simulink library "outp"  (R2021b)
(part 7 of 10)

      link override Signal_Override/_ovrdflg: Value=KOUTP_RUNTM_s_ovrdflg
      link override Signal_Override/_ovrdval: Value=KOUTP_RUNTM_s_ovrdval
  VDID_ResetCDEODTR_km_Inproc : FVT_lib/outp/OverrideAndLimit  SystemSampleTime=-1  VariantActivationTime=update diagram  Latency=0  AutoFrameSizeCalculation=off
      link override Signal_Limit/_maxval: Value=KOUTP_ResetCDEODTR_km_maxval
      link override Signal_Limit/_minval: Value=KOUTP_ResetCDEODTR_km_minval
      link override Signal_Override/_ovrdflg: Value=KOUTP_ResetCDEODTR_km_ovrdflg
      link override Signal_Override/_ovrdval: Value=KOUTP_ResetCDEODTR_km_ovrdval
  VDID_STASUP_enum_Inproc : FVT_lib/outp/OverrideAndLimit  SystemSampleTime=-1  VariantActivationTime=update diagram  Latency=0  AutoFrameSizeCalculation=off
      link override Signal_Limit/_maxval: Value=KOUTP_STASUP_enum_maxval
      link override Signal_Limit/_minval: Value=KOUTP_STASUP_enum_minval
      link override Signal_Override/_ovrdflg: Value=KOUTP_STASUP_enum_ovrdflg
      link override Signal_Override/_ovrdval: Value=KOUTP_STASUP_enum_ovrdval
  VDID_TEBPSAL_kWh_Inproc : FVT_lib/outp/OverrideAndLimit  SystemSampleTime=-1  VariantActivationTime=update diagram  Latency=0  AutoFrameSizeCalculation=off
      link override Signal_Limit/_maxval: Value=KOUTP_TEBPSAL_kWh_maxval
      link override Signal_Limit/_minval: Value=KOUTP_TEBPSAL_kWh_minval
      link override Signal_Override/_ovrdflg: Value=KOUTP_TEBPSAL_kWh_ovrdflg
      link override Signal_Override/_ovrdval: Value=KOUTP_TEBPSAL_kWh_ovrdval
  VDID_TEBPSAR_kWh_Inproc : FVT_lib/outp/OverrideAndLimit  SystemSampleTime=-1  VariantActivationTime=update diagram  Latency=0  AutoFrameSizeCalculation=off
      link override Signal_Limit/_maxval: Value=KOUTP_TEBPSAR_kWh_maxval
      link override Signal_Limit/_minval: Value=KOUTP_TEBPSAR_kWh_minval
      link override Signal_Override/_ovrdflg: Value=KOUTP_TEBPSAR_kWh_ovrdflg
      link override Signal_Override/_ovrdval: Value=KOUTP_TEBPSAR_kWh_ovrdval
  VDID_TGEOVCL_kWh_Inproc : FVT_lib/outp/OverrideAndLimit  SystemSampleTime=-1  VariantActivationTime=update diagram  Latency=0  AutoFrameSizeCalculation=off
      link override Signal_Limit/_maxval: Value=KOUTP_TGEOVCL_kWh_maxval
      link override Signal_Limit/_minval: Value=KOUTP_TGEOVCL_kWh_minval
      link override Signal_Override/_ovrdflg: Value=KOUTP_TGEOVCL_kWh_ovrdflg
      link override Signal_Override/_ovrdval: Value=KOUTP_TGEOVCL_kWh_ovrdval
  VDID_TGEOVCR_kWh_Inproc : FVT_lib/outp/OverrideAndLimit  SystemSampleTime=-1  VariantActivationTime=update diagram  Latency=0  AutoFrameSizeCalculation=off
      link override Signal_Limit/_maxval: Value=KOUTP_TGEOVCR_kWh_maxval
      link override Signal_Limit/_minval: Value=KOUTP_TGEOVCR_kWh_minval
      link override Signal_Override/_ovrdflg: Value=KOUTP_TGEOVCR_kWh_ovrdflg
      link override Signal_Override/_ovrdval: Value=KOUTP_TGEOVCR_kWh_ovrdval
  VDID_TNBCPSAL_Ahr_Inproc : FVT_lib/outp/OverrideAndLimit  SystemSampleTime=-1  VariantActivationTime=update diagram  Latency=0  AutoFrameSizeCalculation=off
      link override Signal_Limit/_maxval: Value=KOUTP_TNBCPSAL_Ahr_maxval
      link override Signal_Limit/_minval: Value=KOUTP_TNBCPSAL_Ahr_minval
      link override Signal_Override/_ovrdflg: Value=KOUTP_TNBCPSAL_Ahr_ovrdflg
      link override Signal_Override/_ovrdval: Value=KOUTP_TNBCPSAL_Ahr_ovrdval
  VDID_TNBCPSAR_Ahr_Inproc : FVT_lib/outp/OverrideAndLimit  SystemSampleTime=-1  VariantActivationTime=update diagram  Latency=0  AutoFrameSizeCalculation=off
      link override Signal_Limit/_maxval: Value=KOUTP_TNBCPSAR_Ahr_maxval
      link override Signal_Limit/_minval: Value=KOUTP_TNBCPSAR_Ahr_minval
      link override Signal_Override/_ovrdflg: Value=KOUTP_TNBCPSAR_Ahr_ovrdflg
      link override Signal_Override/_ovrdval: Value=KOUTP_TNBCPSAR_Ahr_ovrdval
  VDID_TNECPSAL_kWh_Inproc : FVT_lib/outp/OverrideAndLimit  SystemSampleTime=-1  VariantActivationTime=update diagram  Latency=0  AutoFrameSizeCalculation=off
      link override Signal_Limit/_maxval: Value=KOUTP_TNECPSAL_kWh_maxval
      link override Signal_Limit/_minval: Value=KOUTP_TNECPSAL_kWh_minval
      link override Signal_Override/_ovrdflg: Value=KOUTP_TNECPSAL_kWh_ovrdflg
      link override Signal_Override/_ovrdval: Value=KOUTP_TNECPSAL_kWh_ovrdval
  VDID_TNECPSAR_kWh_Inproc : FVT_lib/outp/OverrideAndLimit  SystemSampleTime=-1  VariantActivationTime=update diagram  Latency=0  AutoFrameSizeCalculation=off
      link override Signal_Limit/_maxval: Value=KOUTP_TNECPSAR_kWh_maxval
      link override Signal_Limit/_minval: Value=KOUTP_TNECPSAR_kWh_minval
      link override Signal_Override/_ovrdflg: Value=KOUTP_TNECPSAR_kWh_ovrdflg
      link override Signal_Override/_ovrdval: Value=KOUTP_TNECPSAR_kWh_ovrdval
  VDID_VSS_kph_Inproc : FVT_lib/outp/OverrideAndLimit  SystemSampleTime=-1  VariantActivationTime=update diagram  Latency=0  AutoFrameSizeCalculation=off
      link override Signal_Limit/_maxval: Value=KOUTP_VSS_kph_maxval
      link override Signal_Limit/_minval: Value=KOUTP_VSS_kph_minval
      link override Signal_Override/_ovrdflg: Value=KOUTP_VSS_kph_ovrdflg
      link override Signal_Override/_ovrdval: Value=KOUTP_VSS_kph_ovrdval
  VDID_VinCode_cnt_Inproc : FVT_lib/outp/OverrideAndLimit  SystemSampleTime=-1  VariantActivationTime=update diagram  Latency=0  AutoFrameSizeCalculation=off
      link override Signal_Limit/_maxval: Value=KOUTP_VinCode_cnt_maxval
      link override Signal_Limit/_minval: Value=KOUTP_VinCode_cnt_minval
      link override Signal_Override/_ovrdflg: Value=KOUTP_VinCode_cnt_ovrdflg
      link override Signal_Override/_ovrdval: Value=KOUTP_VinCode_cnt_ovrdval
  VDID_WARMUPS_cnt_Inproc : FVT_lib/outp/OverrideAndLimit  SystemSampleTime=-1  VariantActivationTime=update diagram  Latency=0  AutoFrameSizeCalculation=off
      link override Signal_Limit/_maxval: Value=KOUTP_WARMUPS_cnt_maxval
      link override Signal_Limit/_minval: Value=KOUTP_WARMUPS_cnt_minval
      link override Signal_Override/_ovrdflg: Value=KOUTP_WARMUPS_cnt_ovrdflg
      link override Signal_Override/_ovrdval: Value=KOUTP_WARMUPS_cnt_ovrdval
  VDKC_DKCAuthSta_enum_Inproc : FVT_lib/outp/OverrideAndLimit  SystemSampleTime=-1  VariantActivationTime=update diagram  Latency=0  AutoFrameSizeCalculation=off
      link override Signal_Limit/_maxval: Value=KOUTP_DKCAuthSta_enum_maxval
      link override Signal_Limit/_minval: Value=KOUTP_DKCAuthSta_enum_minval
      link override Signal_Override/_ovrdflg: Value=KOUTP_DKCAuthSta_enum_ovrdflg
      link override Signal_Override/_ovrdval: Value=KOUTP_DKCAuthSta_enum_ovrdval
  VDKC_DKCTimeSN_cnt_Inproc : FVT_lib/outp/OverrideAndLimit  SystemSampleTime=-1  VariantActivationTime=update diagram  Latency=0  AutoFrameSizeCalculation=off
      link override Signal_Limit/_maxval: Value=KOUTP_DKCTimeSN_cnt_maxval
      link override Signal_Limit/_minval: Value=KOUTP_DKCTimeSN_cnt_minval
      link override Signal_Override/_ovrdflg: Value=KOUTP_DKCTimeSN_cnt_ovrdflg
      link override Signal_Override/_ovrdval: Value=KOUTP_DKCTimeSN_cnt_ovrdval
  VDKC_DKeyWelcomeSta_enum_Inproc : FVT_lib/outp/OverrideAndLimit  SystemSampleTime=-1  VariantActivationTime=update diagram  Latency=0  AutoFrameSizeCalculation=off
      link override Signal_Limit/_maxval: Value=KOUTP_DKeyWelcomeSta_enum_maxval
      link override Signal_Limit/_minval: Value=KOUTP_DKeyWelcomeSta_enum_minval
      link override Signal_Override/_ovrdflg: Value=KOUTP_DKeyWelcomeSta_enum_ovrdflg
      link override Signal_Override/_ovrdval: Value=KOUTP_DKeyWelcomeSta_enum_ovrdval
  VDKC_DkeyAreaRAPSSta_enum_Inproc : FVT_lib/outp/OverrideAndLimit  SystemSampleTime=-1  VariantActivationTime=update diagram  Latency=0  AutoFrameSizeCalculation=off
      link override Signal_Limit/_maxval: Value=KOUTP_DkeyAreaRAPSSta_enum_maxval
      link override Signal_Limit/_minval: Value=KOUTP_DkeyAreaRAPSSta_enum_minval
      link override Signal_Override/_ovrdflg: Value=KOUTP_DkeyAreaRAPSSta_enum_ovrdflg
      link override Signal_Override/_ovrdval: Value=KOUTP_DkeyAreaRAPSSta_enum_ovrdval
  VDKC_DkeyShowIVISta_enum_Inproc : FVT_lib/outp/OverrideAndLimit  SystemSampleTime=-1  VariantActivationTime=update diagram  Latency=0  AutoFrameSizeCalculation=off
      link override Signal_Limit/_maxval: Value=KOUTP_DkeyShowIVISta_enum_maxval
      link override Signal_Limit/_minval: Value=KOUTP_DkeyShowIVISta_enum_minval
      link override Signal_Override/_ovrdflg: Value=KOUTP_DkeyShowIVISta_enum_ovrdflg
      link override Signal_Override/_ovrdval: Value=KOUTP_DkeyShowIVISta_enum_ovrdval
  VDKC_FDCDKCAllowSleep_flg_Inproc : FVT_lib/outp/OverrideAndLimit  SystemSampleTime=-1  VariantActivationTime=update diagram  Latency=0  AutoFrameSizeCalculation=off
      link override Signal_Limit/_maxval: Value=KOUTP_FDCDKCAllowSleep_flg_maxval
      link override Signal_Limit/_minval: Value=KOUTP_FDCDKCAllowSleep_flg_minval
      link override Signal_Override/_ovrdflg: Value=KOUTP_FDCDKCAllowSleep_flg_ovrdflg
      link override Signal_Override/_ovrdval: Value=KOUTP_FDCDKCAllowSleep_flg_ovrdval
  VDKC_JudgeKeepUnlockZone_flg_Inproc : FVT_lib/outp/OverrideAndLimit  SystemSampleTime=-1  VariantActivationTime=update diagram  Latency=0  AutoFrameSizeCalculation=off
      link override Signal_Limit/_maxval: Value=KOUTP_JudgeKeepUnlockZone_flg_maxval
      link override Signal_Limit/_minval: Value=KOUTP_JudgeKeepUnlockZone_flg_minval
      link override Signal_Override/_ovrdflg: Value=KOUTP_JudgeKeepUnlockZone_flg_ovrdflg
      link override Signal_Override/_ovrdval: Value=KOUTP_JudgeKeepUnlockZone_flg_ovrdval
  VDKC_KeyAreaLockUnlock_enum_Inproc : FVT_lib/outp/OverrideAndLimit  SystemSampleTime=-1  VariantActivationTime=update diagram  Latency=0  AutoFrameSizeCalculation=off
      link override Signal_Limit/_maxval: Value=KOUTP_KeyAreaLockUnlock_enum_maxval
      link override Signal_Limit/_minval: Value=KOUTP_KeyAreaLockUnlock_enum_minval
      link override Signal_Override/_ovrdflg: Value=KOUTP_KeyAreaLockUnlock_enum_ovrdflg
      link override Signal_Override/_ovrdval: Value=KOUTP_KeyAreaLockUnlock_enum_ovrdval
  VDKC_KeyAreaPS_enum_Inproc : FVT_lib/outp/OverrideAndLimit  SystemSampleTime=-1  VariantActivationTime=update diagram  Latency=0  AutoFrameSizeCalculation=off
      link override Signal_Limit/_maxval: Value=KOUTP_KeyAreaPS_enum_maxval
      link override Signal_Limit/_minval: Value=KOUTP_KeyAreaPS_enum_minval
      link override Signal_Override/_ovrdflg: Value=KOUTP_KeyAreaPS_enum_ovrdflg
      link override Signal_Override/_ovrdval: Value=KOUTP_KeyAreaPS_enum_ovrdval
  VDKC_KeyAreaPTG_enum_Inproc : FVT_lib/outp/OverrideAndLimit  SystemSampleTime=-1  VariantActivationTime=update diagram  Latency=0  AutoFrameSizeCalculation=off
      link override Signal_Limit/_maxval: Value=KOUTP_KeyAreaPTG_enum_maxval
      link override Signal_Limit/_minval: Value=KOUTP_KeyAreaPTG_enum_minval
      link override Signal_Override/_ovrdflg: Value=KOUTP_KeyAreaPTG_enum_ovrdflg
      link override Signal_Override/_ovrdval: Value=KOUTP_KeyAreaPTG_enum_ovrdval
  VDKC_KeyAreaSPTGSta_enum_Inproc : FVT_lib/outp/OverrideAndLimit  SystemSampleTime=-1  VariantActivationTime=update diagram  Latency=0  AutoFrameSizeCalculation=off
      link override Signal_Limit/_maxval: Value=KOUTP_KeyAreaSPTGSta_enum_maxval
      link override Signal_Limit/_minval: Value=KOUTP_KeyAreaSPTGSta_enum_minval
      link override Signal_Override/_ovrdflg: Value=KOUTP_KeyAreaSPTGSta_enum_ovrdflg
      link override Signal_Override/_ovrdval: Value=KOUTP_KeyAreaSPTGSta_enum_ovrdval
  VDKC_KeyMissSta_flg_Inproc : FVT_lib/outp/OverrideAndLimit  SystemSampleTime=-1  VariantActivationTime=update diagram  Latency=0  AutoFrameSizeCalculation=off
      link override Signal_Limit/_maxval: Value=KOUTP_KeyMissSta_flg_maxval
      link override Signal_Limit/_minval: Value=KOUTP_KeyMissSta_flg_minval
      link override Signal_Override/_ovrdflg: Value=KOUTP_KeyMissSta_flg_ovrdflg
      link override Signal_Override/_ovrdval: Value=KOUTP_KeyMissSta_flg_ovrdval
  VDKC_KeyModeSta_enum_Inproc : FVT_lib/outp/OverrideAndLimit  SystemSampleTime=-1  VariantActivationTime=update diagram  Latency=0  AutoFrameSizeCalculation=off
      link override Signal_Limit/_maxval: Value=KOUTP_KeyModeSta_enum_maxval
      link override Signal_Limit/_minval: Value=KOUTP_KeyModeSta_enum_minval
      link override Signal_Override/_ovrdflg: Value=KOUTP_KeyModeSta_enum_ovrdflg
      link override Signal_Override/_ovrdval: Value=KOUTP_KeyModeSta_enum_ovrdval
  VDKC_KeyNumSta_enum_Inproc : FVT_lib/outp/OverrideAndLimit  SystemSampleTime=-1  VariantActivationTime=update diagram  Latency=0  AutoFrameSizeCalculation=off
      link override Signal_Limit/_maxval: Value=KOUTP_KeyNumSta_enum_maxval
      link override Signal_Limit/_minval: Value=KOUTP_KeyNumSta_enum_minval
      link override Signal_Override/_ovrdflg: Value=KOUTP_KeyNumSta_enum_ovrdflg
      link override Signal_Override/_ovrdval: Value=KOUTP_KeyNumSta_enum_ovrdval
  VDKC_KeyTypeSta_enum_Inproc : FVT_lib/outp/OverrideAndLimit  SystemSampleTime=-1  VariantActivationTime=update diagram  Latency=0  AutoFrameSizeCalculation=off
      link override Signal_Limit/_maxval: Value=KOUTP_KeyTypeSta_enum_maxval
      link override Signal_Limit/_minval: Value=KOUTP_KeyTypeSta_enum_minval
      link override Signal_Override/_ovrdflg: Value=KOUTP_KeyTypeSta_enum_ovrdflg
      link override Signal_Override/_ovrdval: Value=KOUTP_KeyTypeSta_enum_ovrdval
  VDKC_PCommandToBCM_enum_Inproc : FVT_lib/outp/OverrideAndLimit  SystemSampleTime=-1  VariantActivationTime=update diagram  Latency=0  AutoFrameSizeCalculation=off
      link override Signal_Limit/_maxval: Value=KOUTP_PCommandToBCM_enum_maxval
      link override Signal_Limit/_minval: Value=KOUTP_PCommandToBCM_enum_minval
      link override Signal_Override/_ovrdflg: Value=KOUTP_PCommandToBCM_enum_ovrdflg
      link override Signal_Override/_ovrdval: Value=KOUTP_PCommandToBCM_enum_ovrdval
  VDKC_ParkingModeCmd_enum_Inproc : FVT_lib/outp/OverrideAndLimit  SystemSampleTime=-1  VariantActivationTime=update diagram  Latency=0  AutoFrameSizeCalculation=off
      link override Signal_Limit/_maxval: Value=KOUTP_ParkingModeCmd_enum_maxval
      link override Signal_Limit/_minval: Value=KOUTP_ParkingModeCmd_enum_minval
      link override Signal_Override/_ovrdflg: Value=KOUTP_ParkingModeCmd_enum_ovrdflg
      link override Signal_Override/_ovrdval: Value=KOUTP_ParkingModeCmd_enum_ovrdval
  VDKC_TimeSNDKCFbk_cnt_Inproc : FVT_lib/outp/OverrideAndLimit  SystemSampleTime=-1  VariantActivationTime=update diagram  Latency=0  AutoFrameSizeCalculation=off
      link override Signal_Limit/_maxval: Value=KOUTP_TimeSNDKCFbk_cnt_maxval
      link override Signal_Limit/_minval: Value=KOUTP_TimeSNDKCFbk_cnt_minval
      link override Signal_Override/_ovrdflg: Value=KOUTP_TimeSNDKCFbk_cnt_ovrdflg
      link override Signal_Override/_ovrdval: Value=KOUTP_TimeSNDKCFbk_cnt_ovrdval
  VDKC_UIDLowPowerSta_enum_Inproc : FVT_lib/outp/OverrideAndLimit  SystemSampleTime=-1  VariantActivationTime=update diagram  Latency=0  AutoFrameSizeCalculation=off
      link override Signal_Limit/_maxval: Value=KOUTP_UIDLowPowerSta_enum_maxval
      link override Signal_Limit/_minval: Value=KOUTP_UIDLowPowerSta_enum_minval
      link override Signal_Override/_ovrdflg: Value=KOUTP_UIDLowPowerSta_enum_ovrdflg
      link override Signal_Override/_ovrdval: Value=KOUTP_UIDLowPowerSta_enum_ovrdval
  VDSC_DISCButtSta_flg_Inproc : FVT_lib/outp/OverrideAndLimit  SystemSampleTime=-1  VariantActivationTime=update diagram  Latency=0  AutoFrameSizeCalculation=off
      link override Signal_Limit/_maxval: Value=KOUTP_DISCButtSta_flg_maxval
      link override Signal_Limit/_minval: Value=KOUTP_DISCButtSta_flg_minval
      link override Signal_Override/_ovrdflg: Value=KOUTP_DISCButtSta_flg_ovrdflg
      link override Signal_Override/_ovrdval: Value=KOUTP_DISCButtSta_flg_ovrdval
  VDSC_DISCSta_enum_Inproc : FVT_lib/outp/OverrideAndLimit  SystemSampleTime=-1  VariantActivationTime=update diagram  Latency=0  AutoFrameSizeCalculation=off
      link override Signal_Limit/_maxval: Value=KOUTP_DISCSta_enum_maxval
      link override Signal_Limit/_minval: Value=KOUTP_DISCSta_enum_minval
      link override Signal_Override/_ovrdflg: Value=KOUTP_DISCSta_enum_ovrdflg
      link override Signal_Override/_ovrdval: Value=KOUTP_DISCSta_enum_ovrdval
  VDSC_DISCTargetSpd_kph_Inproc : FVT_lib/outp/OverrideAndLimit  SystemSampleTime=-1  VariantActivationTime=update diagram  Latency=0  AutoFrameSizeCalculation=off
      link override Signal_Limit/_maxval: Value=KOUTP_DISCTargetSpd_kph_maxval
      link override Signal_Limit/_minval: Value=KOUTP_DISCTargetSpd_kph_minval
      link override Signal_Override/_ovrdflg: Value=KOUTP_DISCTargetSpd_kph_ovrdflg
      link override Signal_Override/_ovrdval: Value=KOUTP_DISCTargetSpd_kph_ovrdval
  VDSC_DISCTurn_flg_Inproc : FVT_lib/outp/OverrideAndLimit  SystemSampleTime=-1  VariantActivationTime=update diagram  Latency=0  AutoFrameSizeCalculation=off
      link override Signal_Limit/_maxval: Value=KOUTP_DISCTurn_flg_maxval
      link override Signal_Limit/_minval: Value=KOUTP_DISCTurn_flg_minval
      link override Signal_Override/_ovrdflg: Value=KOUTP_DISCTurn_flg_ovrdflg
      link override Signal_Override/_ovrdval: Value=KOUTP_DISCTurn_flg_ovrdval
  VNMM_ActiveWU_flg_Inproc : FVT_lib/outp/OverrideAndLimit  SystemSampleTime=-1  VariantActivationTime=update diagram  Latency=0  AutoFrameSizeCalculation=off
      link override Signal_Limit/_maxval: Value=KOUTP_ActiveWU_flg_maxval
      link override Signal_Limit/_minval: Value=KOUTP_ActiveWU_flg_minval
      link override Signal_Override/_ovrdflg: Value=KOUTP_ActiveWU_flg_ovrdflg
      link override Signal_Override/_ovrdval: Value=KOUTP_ActiveWU_flg_ovrdval
  VNMM_AllCANTxReq_flg_Inproc : FVT_lib/outp/OverrideAndLimit  SystemSampleTime=-1  VariantActivationTime=update diagram  Latency=0  AutoFrameSizeCalculation=off
      link override Signal_Limit/_maxval: Value=KOUTP_AllCANTxReq_flg_maxval
      link override Signal_Limit/_minval: Value=KOUTP_AllCANTxReq_flg_minval
      link override Signal_Override/_ovrdflg: Value=KOUTP_AllCANTxReq_flg_ovrdflg
      link override Signal_Override/_ovrdval: Value=KOUTP_AllCANTxReq_flg_ovrdval
  VNMM_Awake_enum_Inproc : FVT_lib/outp/OverrideAndLimit  SystemSampleTime=-1  VariantActivationTime=update diagram  Latency=0  AutoFrameSizeCalculation=off
      link override Signal_Limit/_maxval: Value=KOUTP_Awake_enum_maxval
      link override Signal_Limit/_minval: Value=KOUTP_Awake_enum_minval
      link override Signal_Override/_ovrdflg: Value=KOUTP_Awake_enum_ovrdflg
      link override Signal_Override/_ovrdval: Value=KOUTP_Awake_enum_ovrdval
  VNMM_CSB_flg_Inproc : FVT_lib/outp/OverrideAndLimit  SystemSampleTime=-1  VariantActivationTime=update diagram  Latency=0  AutoFrameSizeCalculation=off
      link override Signal_Limit/_maxval: Value=KOUTP_CSB_flg_maxval
      link override Signal_Limit/_minval: Value=KOUTP_CSB_flg_minval
      link override Signal_Override/_ovrdflg: Value=KOUTP_CSB_flg_ovrdflg
      link override Signal_Override/_ovrdval: Value=KOUTP_CSB_flg_ovrdval
  VNMM_ErrorState_enum_Inproc : FVT_lib/outp/OverrideAndLimit  SystemSampleTime=-1  VariantActivationTime=update diagram  Latency=0  AutoFrameSizeCalculation=off
      link override Signal_Limit/_maxval: Value=KOUTP_ErrorState_enum_maxval
      link override Signal_Limit/_minval: Value=KOUTP_ErrorState_enum_minval
      link override Signal_Override/_ovrdflg: Value=KOUTP_ErrorState_enum_ovrdflg
      link override Signal_Override/_ovrdval: Value=KOUTP_ErrorState_enum_ovrdval
  VNMM_NMmTxReq_flg_Inproc : FVT_lib/outp/OverrideAndLimit  SystemSampleTime=-1  VariantActivationTime=update diagram  Latency=0  AutoFrameSizeCalculation=off
      link override Signal_Limit/_maxval: Value=KOUTP_NMmTxReq_flg_maxval
      link override Signal_Limit/_minval: Value=KOUTP_NMmTxReq_flg_minval
      link override Signal_Override/_ovrdflg: Value=KOUTP_NMmTxReq_flg_ovrdflg
      link override Signal_Override/_ovrdval: Value=KOUTP_NMmTxReq_flg_ovrdval
  VNMM_NetworkReq_flg_Inproc : FVT_lib/outp/OverrideAndLimit  SystemSampleTime=-1  VariantActivationTime=update diagram  Latency=0  AutoFrameSizeCalculation=off
      link override Signal_Limit/_maxval: Value=KOUTP_NetworkReq_flg_maxval
      link override Signal_Limit/_minval: Value=KOUTP_NetworkReq_flg_minval
      link override Signal_Override/_ovrdflg: Value=KOUTP_NetworkReq_flg_ovrdflg
      link override Signal_Override/_ovrdval: Value=KOUTP_NetworkReq_flg_ovrdval
  VNMM_NodeID_enum_Inproc : FVT_lib/outp/OverrideAndLimit  SystemSampleTime=-1  VariantActivationTime=update diagram  Latency=0  AutoFrameSizeCalculation=off
      link override Signal_Limit/_maxval: Value=KOUTP_NodeID_enum_maxval
      link override Signal_Limit/_minval: Value=KOUTP_NodeID_enum_minval
      link override Signal_Override/_ovrdflg: Value=KOUTP_NodeID_enum_ovrdflg
      link override Signal_Override/_ovrdval: Value=KOUTP_NodeID_enum_ovrdval
  VNMM_PNI_flg_Inproc : FVT_lib/outp/OverrideAndLimit  SystemSampleTime=-1  VariantActivationTime=update diagram  Latency=0  AutoFrameSizeCalculation=off
      link override Signal_Limit/_maxval: Value=KOUTP_PNI_flg_maxval
      link override Signal_Limit/_minval: Value=KOUTP_PNI_flg_minval
      link override Signal_Override/_ovrdflg: Value=KOUTP_PNI_flg_ovrdflg
      link override Signal_Override/_ovrdval: Value=KOUTP_PNI_flg_ovrdval
  VNMM_RptMsgReq_flg_Inproc : FVT_lib/outp/OverrideAndLimit  SystemSampleTime=-1  VariantActivationTime=update diagram  Latency=0  AutoFrameSizeCalculation=off
      link override Signal_Limit/_maxval: Value=KOUTP_RptMsgReq_flg_maxval
      link override Signal_Limit/_minval: Value=KOUTP_RptMsgReq_flg_minval
      link override Signal_Override/_ovrdflg: Value=KOUTP_RptMsgReq_flg_ovrdflg
      link override Signal_Override/_ovrdval: Value=KOUTP_RptMsgReq_flg_ovrdval
  VNMM_SysNMmSta_enum_Inproc : FVT_lib/outp/OverrideAndLimit  SystemSampleTime=-1  VariantActivationTime=update diagram  Latency=0  AutoFrameSizeCalculation=off
      link override Signal_Limit/_maxval: Value=KOUTP_SysNMmSta_enum_maxval
      link override Signal_Limit/_minval: Value=KOUTP_SysNMmSta_enum_minval
      link override Signal_Override/_ovrdflg: Value=KOUTP_SysNMmSta_enum_ovrdflg
      link override Signal_Override/_ovrdval: Value=KOUTP_SysNMmSta_enum_ovrdval
  VNMM_WakeUp_enum_Inproc : FVT_lib/outp/OverrideAndLimit  SystemSampleTime=-1  VariantActivationTime=update diagram  Latency=0  AutoFrameSizeCalculation=off
      link override Signal_Limit/_maxval: Value=KOUTP_WakeUp_enum_maxval
      link override Signal_Limit/_minval: Value=KOUTP_WakeUp_enum_minval
      link override Signal_Override/_ovrdflg: Value=KOUTP_WakeUp_enum_ovrdflg
      link override Signal_Override/_ovrdval: Value=KOUTP_WakeUp_enum_ovrdval
  VPMM_ACHVLoopDem_enum_Inproc : FVT_lib/outp/OverrideAndLimit  SystemSampleTime=-1  VariantActivationTime=update diagram  Latency=0  AutoFrameSizeCalculation=off
      link override Signal_Limit/_maxval: Value=KOUTP_ACHVLoopDem_enum_maxval
      link override Signal_Limit/_minval: Value=KOUTP_ACHVLoopDem_enum_minval
      link override Signal_Override/_ovrdflg: Value=KOUTP_ACHVLoopDem_enum_ovrdflg
      link override Signal_Override/_ovrdval: Value=KOUTP_ACHVLoopDem_enum_ovrdval
  VPMM_ActiveDischargeReq_enum_Inproc : FVT_lib/outp/OverrideAndLimit  SystemSampleTime=-1  VariantActivationTime=update diagram  Latency=0  AutoFrameSizeCalculation=off
      link override Signal_Limit/_maxval: Value=KOUTP_ActiveDischargeReq_enum_maxval
      link override Signal_Limit/_minval: Value=KOUTP_ActiveDischargeReq_enum_minval
      link override Signal_Override/_ovrdflg: Value=KOUTP_ActiveDischargeReq_enum_ovrdflg
      link override Signal_Override/_ovrdval: Value=KOUTP_ActiveDischargeReq_enum_ovrdval
  VPMM_BattHVDem_enum_Inproc : FVT_lib/outp/OverrideAndLimit  SystemSampleTime=-1  VariantActivationTime=update diagram  Latency=0  AutoFrameSizeCalculation=off
      link override Signal_Limit/_maxval: Value=KOUTP_BattHVDem_enum_maxval
      link override Signal_Limit/_minval: Value=KOUTP_BattHVDem_enum_minval
      link override Signal_Override/_ovrdflg: Value=KOUTP_BattHVDem_enum_ovrdflg
      link override Signal_Override/_ovrdval: Value=KOUTP_BattHVDem_enum_ovrdval
  VPMM_CACRlyDem_enum_Inproc : FVT_lib/outp/OverrideAndLimit  SystemSampleTime=-1  VariantActivationTime=update diagram  Latency=0  AutoFrameSizeCalculation=off
      link override Signal_Limit/_maxval: Value=KOUTP_CACRlyDem_enum_maxval
      link override Signal_Limit/_minval: Value=KOUTP_CACRlyDem_enum_minval
      link override Signal_Override/_ovrdflg: Value=KOUTP_CACRlyDem_enum_ovrdflg
      link override Signal_Override/_ovrdval: Value=KOUTP_CACRlyDem_enum_ovrdval
  VPMM_ChrgBCUHVFail_flg_Inproc : FVT_lib/outp/OverrideAndLimit  SystemSampleTime=-1  VariantActivationTime=update diagram  Latency=0  AutoFrameSizeCalculation=off
      link override Signal_Limit/_maxval: Value=KOUTP_ChrgBCUHVFail_flg_maxval
      link override Signal_Limit/_minval: Value=KOUTP_ChrgBCUHVFail_flg_minval
      link override Signal_Override/_ovrdflg: Value=KOUTP_ChrgBCUHVFail_flg_ovrdflg
      link override Signal_Override/_ovrdval: Value=KOUTP_ChrgBCUHVFail_flg_ovrdval
  VPMM_ChrgFault_enum_Inproc : FVT_lib/outp/OverrideAndLimit  SystemSampleTime=-1  VariantActivationTime=update diagram  Latency=0  AutoFrameSizeCalculation=off
      link override Signal_Limit/_maxval: Value=KOUTP_ChrgFault_enum_maxval
      link override Signal_Limit/_minval: Value=KOUTP_ChrgFault_enum_minval
      link override Signal_Override/_ovrdflg: Value=KOUTP_ChrgFault_enum_ovrdflg
      link override Signal_Override/_ovrdval: Value=KOUTP_ChrgFault_enum_ovrdval
  VPMM_ChrgPowerUpFail_flg_Inproc : FVT_lib/outp/OverrideAndLimit  SystemSampleTime=-1  VariantActivationTime=update diagram  Latency=0  AutoFrameSizeCalculation=off
      link override Signal_Limit/_maxval: Value=KOUTP_ChrgPowerUpFail_flg_maxval
      link override Signal_Limit/_minval: Value=KOUTP_ChrgPowerUpFail_flg_minval
      link override Signal_Override/_ovrdflg: Value=KOUTP_ChrgPowerUpFail_flg_ovrdflg
      link override Signal_Override/_ovrdval: Value=KOUTP_ChrgPowerUpFail_flg_ovrdval
  VPMM_ChrgState_enum_Inproc : FVT_lib/outp/OverrideAndLimit  SystemSampleTime=-1  VariantActivationTime=update diagram  Latency=0  AutoFrameSizeCalculation=off
      link override Signal_Limit/_maxval: Value=KOUTP_ChrgState_enum_maxval
      link override Signal_Limit/_minval: Value=KOUTP_ChrgState_enum_minval
      link override Signal_Override/_ovrdflg: Value=KOUTP_ChrgState_enum_ovrdflg
      link override Signal_Override/_ovrdval: Value=KOUTP_ChrgState_enum_ovrdval
  VPMM_DCCurr_A_Inproc : FVT_lib/outp/OverrideAndLimit  SystemSampleTime=-1  VariantActivationTime=update diagram  Latency=0  AutoFrameSizeCalculation=off
      link override Signal_Limit/_maxval: Value=KOUTP_DCCurr_A_maxval
      link override Signal_Limit/_minval: Value=KOUTP_DCCurr_A_minval
      link override Signal_Override/_ovrdflg: Value=KOUTP_DCCurr_A_ovrdflg
      link override Signal_Override/_ovrdval: Value=KOUTP_DCCurr_A_ovrdval
  VPMM_DCDCRlyDem_enum_Inproc : FVT_lib/outp/OverrideAndLimit  SystemSampleTime=-1  VariantActivationTime=update diagram  Latency=0  AutoFrameSizeCalculation=off
      link override Signal_Limit/_maxval: Value=KOUTP_DCDCRlyDem_enum_maxval
      link override Signal_Limit/_minval: Value=KOUTP_DCDCRlyDem_enum_minval
      link override Signal_Override/_ovrdflg: Value=KOUTP_DCDCRlyDem_enum_ovrdflg
      link override Signal_Override/_ovrdval: Value=KOUTP_DCDCRlyDem_enum_ovrdval
  VPMM_DCVol_V_Inproc : FVT_lib/outp/OverrideAndLimit  SystemSampleTime=-1  VariantActivationTime=update diagram  Latency=0  AutoFrameSizeCalculation=off
      link override Signal_Limit/_maxval: Value=KOUTP_DCVol_V_maxval
      link override Signal_Limit/_minval: Value=KOUTP_DCVol_V_minval
      link override Signal_Override/_ovrdflg: Value=KOUTP_DCVol_V_ovrdflg
      link override Signal_Override/_ovrdval: Value=KOUTP_DCVol_V_ovrdval
  VPMM_DrivelineRelease_enum_Inproc : FVT_lib/outp/OverrideAndLimit  SystemSampleTime=-1  VariantActivationTime=update diagram  Latency=0  AutoFrameSizeCalculation=off
      link override Signal_Limit/_maxval: Value=KOUTP_DrivelineRelease_enum_maxval
      link override Signal_Limit/_minval: Value=KOUTP_DrivelineRelease_enum_minval
      link override Signal_Override/_ovrdflg: Value=KOUTP_DrivelineRelease_enum_ovrdflg
      link override Signal_Override/_ovrdval: Value=KOUTP_DrivelineRelease_enum_ovrdval
  VPMM_EHPSRlyDem_enum_Inproc : FVT_lib/outp/OverrideAndLimit  SystemSampleTime=-1  VariantActivationTime=update diagram  Latency=0  AutoFrameSizeCalculation=off
      link override Signal_Limit/_maxval: Value=KOUTP_EHPSRlyDem_enum_maxval
      link override Signal_Limit/_minval: Value=KOUTP_EHPSRlyDem_enum_minval
      link override Signal_Override/_ovrdflg: Value=KOUTP_EHPSRlyDem_enum_ovrdflg
      link override Signal_Override/_ovrdval: Value=KOUTP_EHPSRlyDem_enum_ovrdval
  VPMM_FogTMSRlyCMD_enum_Inproc : FVT_lib/outp/OverrideAndLimit  SystemSampleTime=-1  VariantActivationTime=update diagram  Latency=0  AutoFrameSizeCalculation=off
      link override Signal_Limit/_maxval: Value=KOUTP_FogTMSRlyCMD_enum_maxval
      link override Signal_Limit/_minval: Value=KOUTP_FogTMSRlyCMD_enum_minval
      link override Signal_Override/_ovrdflg: Value=KOUTP_FogTMSRlyCMD_enum_ovrdflg
      link override Signal_Override/_ovrdval: Value=KOUTP_FogTMSRlyCMD_enum_ovrdval
  VPMM_HVFailureChkPass_flg_Inproc : FVT_lib/outp/OverrideAndLimit  SystemSampleTime=-1  VariantActivationTime=update diagram  Latency=0  AutoFrameSizeCalculation=off
      link override Signal_Limit/_maxval: Value=KOUTP_HVFailureChkPass_flg_maxval
      link override Signal_Limit/_minval: Value=KOUTP_HVFailureChkPass_flg_minval
      link override Signal_Override/_ovrdflg: Value=KOUTP_HVFailureChkPass_flg_ovrdflg
      link override Signal_Override/_ovrdval: Value=KOUTP_HVFailureChkPass_flg_ovrdval
  VPMM_HVILDetectFail_flg_Inproc : FVT_lib/outp/OverrideAndLimit  SystemSampleTime=-1  VariantActivationTime=update diagram  Latency=0  AutoFrameSizeCalculation=off
      link override Signal_Limit/_maxval: Value=KOUTP_HVILDetectFail_flg_maxval
      link override Signal_Limit/_minval: Value=KOUTP_HVILDetectFail_flg_minval
      link override Signal_Override/_ovrdflg: Value=KOUTP_HVILDetectFail_flg_ovrdflg
      link override Signal_Override/_ovrdval: Value=KOUTP_HVILDetectFail_flg_ovrdval
  VPMM_HVILFail_flg_Inproc : FVT_lib/outp/OverrideAndLimit  SystemSampleTime=-1  VariantActivationTime=update diagram  Latency=0  AutoFrameSizeCalculation=off
      link override Signal_Limit/_maxval: Value=KOUTP_HVILFail_flg_maxval
      link override Signal_Limit/_minval: Value=KOUTP_HVILFail_flg_minval
      link override Signal_Override/_ovrdflg: Value=KOUTP_HVILFail_flg_ovrdflg
      link override Signal_Override/_ovrdval: Value=KOUTP_HVILFail_flg_ovrdval
  VPMM_HVSysReady_enum_Inproc : FVT_lib/outp/OverrideAndLimit  SystemSampleTime=-1  VariantActivationTime=update diagram  Latency=0  AutoFrameSizeCalculation=off
      link override Signal_Limit/_maxval: Value=KOUTP_HVSysReady_enum_maxval
      link override Signal_Limit/_minval: Value=KOUTP_HVSysReady_enum_minval
      link override Signal_Override/_ovrdflg: Value=KOUTP_HVSysReady_enum_ovrdflg
      link override Signal_Override/_ovrdval: Value=KOUTP_HVSysReady_enum_ovrdval
  VPMM_IGNRlyClose_flg_Inproc : FVT_lib/outp/OverrideAndLimit  SystemSampleTime=-1  VariantActivationTime=update diagram  Latency=0  AutoFrameSizeCalculation=off
      link override Signal_Limit/_maxval: Value=KOUTP_IGNRlyClose_flg_maxval
      link override Signal_Limit/_minval: Value=KOUTP_IGNRlyClose_flg_minval
      link override Signal_Override/_ovrdflg: Value=KOUTP_IGNRlyClose_flg_ovrdflg
      link override Signal_Override/_ovrdval: Value=KOUTP_IGNRlyClose_flg_ovrdval
  VPMM_IRCRlyClose_flg_Inproc : FVT_lib/outp/OverrideAndLimit  SystemSampleTime=-1  VariantActivationTime=update diagram  Latency=0  AutoFrameSizeCalculation=off
      link override Signal_Limit/_maxval: Value=KOUTP_IRCRlyClose_flg_maxval
      link override Signal_Limit/_minval: Value=KOUTP_IRCRlyClose_flg_minval
      link override Signal_Override/_ovrdflg: Value=KOUTP_IRCRlyClose_flg_ovrdflg
      link override Signal_Override/_ovrdval: Value=KOUTP_IRCRlyClose_flg_ovrdval
  VPMM_LVBattLowInd_enum_Inproc : FVT_lib/outp/OverrideAndLimit  SystemSampleTime=-1  VariantActivationTime=update diagram  Latency=0  AutoFrameSizeCalculation=off
      link override Signal_Limit/_maxval: Value=KOUTP_LVBattLowInd_enum_maxval
      link override Signal_Limit/_minval: Value=KOUTP_LVBattLowInd_enum_minval
      link override Signal_Override/_ovrdflg: Value=KOUTP_LVBattLowInd_enum_ovrdflg
      link override Signal_Override/_ovrdval: Value=KOUTP_LVBattLowInd_enum_ovrdval
  VPMM_LostHVComActivePwrDown_flg_Inproc : FVT_lib/outp/OverrideAndLimit  SystemSampleTime=-1  VariantActivationTime=update diagram  Latency=0  AutoFrameSizeCalculation=off
      link override Signal_Limit/_maxval: Value=KOUTP_LostHVComActivePwrDown_flg_maxval
      link override Signal_Limit/_minval: Value=KOUTP_LostHVComActivePwrDown_flg_minval
      link override Signal_Override/_ovrdflg: Value=KOUTP_LostHVComActivePwrDown_flg_ovrdflg
      link override Signal_Override/_ovrdval: Value=KOUTP_LostHVComActivePwrDown_flg_ovrdval
  VPMM_MCUHVLoopDem_enum_Inproc : FVT_lib/outp/OverrideAndLimit  SystemSampleTime=-1  VariantActivationTime=update diagram  Latency=0  AutoFrameSizeCalculation=off
      link override Signal_Limit/_maxval: Value=KOUTP_MCUHVLoopDem_enum_maxval
      link override Signal_Limit/_minval: Value=KOUTP_MCUHVLoopDem_enum_minval
      link override Signal_Override/_ovrdflg: Value=KOUTP_MCUHVLoopDem_enum_ovrdflg
      link override Signal_Override/_ovrdval: Value=KOUTP_MCUHVLoopDem_enum_ovrdval
  VPMM_PowerDownFault_enum_Inproc : FVT_lib/outp/OverrideAndLimit  SystemSampleTime=-1  VariantActivationTime=update diagram  Latency=0  AutoFrameSizeCalculation=off
      link override Signal_Limit/_maxval: Value=KOUTP_PowerDownFault_enum_maxval
      link override Signal_Limit/_minval: Value=KOUTP_PowerDownFault_enum_minval
      link override Signal_Override/_ovrdflg: Value=KOUTP_PowerDownFault_enum_ovrdflg
      link override Signal_Override/_ovrdval: Value=KOUTP_PowerDownFault_enum_ovrdval
  VPMM_PowerDownState_enum_Inproc : FVT_lib/outp/OverrideAndLimit  SystemSampleTime=-1  VariantActivationTime=update diagram  Latency=0  AutoFrameSizeCalculation=off
      link override Signal_Limit/_maxval: Value=KOUTP_PowerDownState_enum_maxval
      link override Signal_Limit/_minval: Value=KOUTP_PowerDownState_enum_minval
      link override Signal_Override/_ovrdflg: Value=KOUTP_PowerDownState_enum_ovrdflg
      link override Signal_Override/_ovrdval: Value=KOUTP_PowerDownState_enum_ovrdval
  VPMM_PowerUpFault_enum_Inproc : FVT_lib/outp/OverrideAndLimit  SystemSampleTime=-1  VariantActivationTime=update diagram  Latency=0  AutoFrameSizeCalculation=off
      link override Signal_Limit/_maxval: Value=KOUTP_PowerUpFault_enum_maxval
      link override Signal_Limit/_minval: Value=KOUTP_PowerUpFault_enum_minval
      link override Signal_Override/_ovrdflg: Value=KOUTP_PowerUpFault_enum_ovrdflg
      link override Signal_Override/_ovrdval: Value=KOUTP_PowerUpFault_enum_ovrdval
  VPMM_PowerUpState_enum_Inproc : FVT_lib/outp/OverrideAndLimit  SystemSampleTime=-1  VariantActivationTime=update diagram  Latency=0  AutoFrameSizeCalculation=off
      link override Signal_Limit/_maxval: Value=KOUTP_PowerUpState_enum_maxval
      link override Signal_Limit/_minval: Value=KOUTP_PowerUpState_enum_minval
      link override Signal_Override/_ovrdflg: Value=KOUTP_PowerUpState_enum_ovrdflg
      link override Signal_Override/_ovrdval: Value=KOUTP_PowerUpState_enum_ovrdval
  VPMM_SysPowerMode_enum_Inproc : FVT_lib/outp/OverrideAndLimit  SystemSampleTime=-1  VariantActivationTime=update diagram  Latency=0  AutoFrameSizeCalculation=off
      link override Signal_Limit/_maxval: Value=KOUTP_SysPowerMode_enum_maxval
      link override Signal_Limit/_minval: Value=KOUTP_SysPowerMode_enum_minval
      link override Signal_Override/_ovrdflg: Value=KOUTP_SysPowerMode_enum_ovrdflg
      link override Signal_Override/_ovrdval: Value=KOUTP_SysPowerMode_enum_ovrdval
  VPMM_V2BACPosRlyFit_enum_Inproc : FVT_lib/outp/OverrideAndLimit  SystemSampleTime=-1  VariantActivationTime=update diagram  Latency=0  AutoFrameSizeCalculation=off
      link override Signal_Limit/_maxval: Value=KOUTP_V2BACPosRlyFit_enum_maxval
      link override Signal_Limit/_minval: Value=KOUTP_V2BACPosRlyFit_enum_minval
      link override Signal_Override/_ovrdflg: Value=KOUTP_V2BACPosRlyFit_enum_ovrdflg
      link override Signal_Override/_ovrdval: Value=KOUTP_V2BACPosRlyFit_enum_ovrdval
  VPMM_V2BACPosRlySta_enum_Inproc : FVT_lib/outp/OverrideAndLimit  SystemSampleTime=-1  VariantActivationTime=update diagram  Latency=0  AutoFrameSizeCalculation=off
      link override Signal_Limit/_maxval: Value=KOUTP_V2BACPosRlySta_enum_maxval
      link override Signal_Limit/_minval: Value=KOUTP_V2BACPosRlySta_enum_minval
      link override Signal_Override/_ovrdflg: Value=KOUTP_V2BACPosRlySta_enum_ovrdflg
      link override Signal_Override/_ovrdval: Value=KOUTP_V2BACPosRlySta_enum_ovrdval
  VPMM_V2BAirPosRlyFit_enum_Inproc : FVT_lib/outp/OverrideAndLimit  SystemSampleTime=-1  VariantActivationTime=update diagram  Latency=0  AutoFrameSizeCalculation=off
      link override Signal_Limit/_maxval: Value=KOUTP_V2BAirPosRlyFit_enum_maxval
      link override Signal_Limit/_minval: Value=KOUTP_V2BAirPosRlyFit_enum_minval
      link override Signal_Override/_ovrdflg: Value=KOUTP_V2BAirPosRlyFit_enum_ovrdflg
      link override Signal_Override/_ovrdval: Value=KOUTP_V2BAirPosRlyFit_enum_ovrdval
  VPMM_V2BAirPosRlySta_enum_Inproc : FVT_lib/outp/OverrideAndLimit  SystemSampleTime=-1  VariantActivationTime=update diagram  Latency=0  AutoFrameSizeCalculation=off
      link override Signal_Limit/_maxval: Value=KOUTP_V2BAirPosRlySta_enum_maxval
      link override Signal_Limit/_minval: Value=KOUTP_V2BAirPosRlySta_enum_minval
      link override Signal_Override/_ovrdflg: Value=KOUTP_V2BAirPosRlySta_enum_ovrdflg
      link override Signal_Override/_ovrdval: Value=KOUTP_V2BAirPosRlySta_enum_ovrdval
  VPMM_V2BAux1OnOff_enum_Inproc : FVT_lib/outp/OverrideAndLimit  SystemSampleTime=-1  VariantActivationTime=update diagram  Latency=0  AutoFrameSizeCalculation=off
      link override Signal_Limit/_maxval: Value=KOUTP_V2BAux1OnOff_enum_maxval
      link override Signal_Limit/_minval: Value=KOUTP_V2BAux1OnOff_enum_minval
      link override Signal_Override/_ovrdflg: Value=KOUTP_V2BAux1OnOff_enum_ovrdflg
      link override Signal_Override/_ovrdval: Value=KOUTP_V2BAux1OnOff_enum_ovrdval
  VPMM_V2BAux1RlyFit_enum_Inproc : FVT_lib/outp/OverrideAndLimit  SystemSampleTime=-1  VariantActivationTime=update diagram  Latency=0  AutoFrameSizeCalculation=off
      link override Signal_Limit/_maxval: Value=KOUTP_V2BAux1RlyFit_enum_maxval
      link override Signal_Limit/_minval: Value=KOUTP_V2BAux1RlyFit_enum_minval
      link override Signal_Override/_ovrdflg: Value=KOUTP_V2BAux1RlyFit_enum_ovrdflg
      link override Signal_Override/_ovrdval: Value=KOUTP_V2BAux1RlyFit_enum_ovrdval
  VPMM_V2BAux1RlySta_enum_Inproc : FVT_lib/outp/OverrideAndLimit  SystemSampleTime=-1  VariantActivationTime=update diagram  Latency=0  AutoFrameSizeCalculation=off
      link override Signal_Limit/_maxval: Value=KOUTP_V2BAux1RlySta_enum_maxval
      link override Signal_Limit/_minval: Value=KOUTP_V2BAux1RlySta_enum_minval
      link override Signal_Override/_ovrdflg: Value=KOUTP_V2BAux1RlySta_enum_ovrdflg
      link override Signal_Override/_ovrdval: Value=KOUTP_V2BAux1RlySta_enum_ovrdval
  VPMM_V2BAux2OnOff_enum_Inproc : FVT_lib/outp/OverrideAndLimit  SystemSampleTime=-1  VariantActivationTime=update diagram  Latency=0  AutoFrameSizeCalculation=off
      link override Signal_Limit/_maxval: Value=KOUTP_V2BAux2OnOff_enum_maxval
      link override Signal_Limit/_minval: Value=KOUTP_V2BAux2OnOff_enum_minval
      link override Signal_Override/_ovrdflg: Value=KOUTP_V2BAux2OnOff_enum_ovrdflg
      link override Signal_Override/_ovrdval: Value=KOUTP_V2BAux2OnOff_enum_ovrdval
  VPMM_V2BAux2RlyFit_enum_Inproc : FVT_lib/outp/OverrideAndLimit  SystemSampleTime=-1  VariantActivationTime=update diagram  Latency=0  AutoFrameSizeCalculation=off
      link override Signal_Limit/_maxval: Value=KOUTP_V2BAux2RlyFit_enum_maxval
      link override Signal_Limit/_minval: Value=KOUTP_V2BAux2RlyFit_enum_minval
      link override Signal_Override/_ovrdflg: Value=KOUTP_V2BAux2RlyFit_enum_ovrdflg
      link override Signal_Override/_ovrdval: Value=KOUTP_V2BAux2RlyFit_enum_ovrdval
  VPMM_V2BAux2RlySta_enum_Inproc : FVT_lib/outp/OverrideAndLimit  SystemSampleTime=-1  VariantActivationTime=update diagram  Latency=0  AutoFrameSizeCalculation=off
      link override Signal_Limit/_maxval: Value=KOUTP_V2BAux2RlySta_enum_maxval
      link override Signal_Limit/_minval: Value=KOUTP_V2BAux2RlySta_enum_minval
      link override Signal_Override/_ovrdflg: Value=KOUTP_V2BAux2RlySta_enum_ovrdflg
      link override Signal_Override/_ovrdval: Value=KOUTP_V2BAux2RlySta_enum_ovrdval
  VPMM_V2BAux3OnOff_enum_Inproc : FVT_lib/outp/OverrideAndLimit  SystemSampleTime=-1  VariantActivationTime=update diagram  Latency=0  AutoFrameSizeCalculation=off
      link override Signal_Limit/_maxval: Value=KOUTP_V2BAux3OnOff_enum_maxval
      link override Signal_Limit/_minval: Value=KOUTP_V2BAux3OnOff_enum_minval
      link override Signal_Override/_ovrdflg: Value=KOUTP_V2BAux3OnOff_enum_ovrdflg
      link override Signal_Override/_ovrdval: Value=KOUTP_V2BAux3OnOff_enum_ovrdval
  VPMM_V2BAux3RlyFit_enum_Inproc : FVT_lib/outp/OverrideAndLimit  SystemSampleTime=-1  VariantActivationTime=update diagram  Latency=0  AutoFrameSizeCalculation=off
      link override Signal_Limit/_maxval: Value=KOUTP_V2BAux3RlyFit_enum_maxval
      link override Signal_Limit/_minval: Value=KOUTP_V2BAux3RlyFit_enum_minval
      link override Signal_Override/_ovrdflg: Value=KOUTP_V2BAux3RlyFit_enum_ovrdflg
      link override Signal_Override/_ovrdval: Value=KOUTP_V2BAux3RlyFit_enum_ovrdval
  VPMM_V2BAux3RlySta_enum_Inproc : FVT_lib/outp/OverrideAndLimit  SystemSampleTime=-1  VariantActivationTime=update diagram  Latency=0  AutoFrameSizeCalculation=off
      link override Signal_Limit/_maxval: Value=KOUTP_V2BAux3RlySta_enum_maxval
      link override Signal_Limit/_minval: Value=KOUTP_V2BAux3RlySta_enum_minval
      link override Signal_Override/_ovrdflg: Value=KOUTP_V2BAux3RlySta_enum_ovrdflg
      link override Signal_Override/_ovrdval: Value=KOUTP_V2BAux3RlySta_enum_ovrdval
  VPMM_V2BAux4RlyFit_enum_Inproc : FVT_lib/outp/OverrideAndLimit  SystemSampleTime=-1  VariantActivationTime=update diagram  Latency=0  AutoFrameSizeCalculation=off
      link override Signal_Limit/_maxval: Value=KOUTP_V2BAux4RlyFit_enum_maxval
      link override Signal_Limit/_minval: Value=KOUTP_V2BAux4RlyFit_enum_minval
      link override Signal_Override/_ovrdflg: Value=KOUTP_V2BAux4RlyFit_enum_ovrdflg
      link override Signal_Override/_ovrdval: Value=KOUTP_V2BAux4RlyFit_enum_ovrdval
  VPMM_V2BAux4RlySta_enum_Inproc : FVT_lib/outp/OverrideAndLimit  SystemSampleTime=-1  VariantActivationTime=update diagram  Latency=0  AutoFrameSizeCalculation=off
      link override Signal_Limit/_maxval: Value=KOUTP_V2BAux4RlySta_enum_maxval
      link override Signal_Limit/_minval: Value=KOUTP_V2BAux4RlySta_enum_minval
      link override Signal_Override/_ovrdflg: Value=KOUTP_V2BAux4RlySta_enum_ovrdflg
      link override Signal_Override/_ovrdval: Value=KOUTP_V2BAux4RlySta_enum_ovrdval
  VPMM_V2BDCDCPosRlyFit_enum_Inproc : FVT_lib/outp/OverrideAndLimit  SystemSampleTime=-1  VariantActivationTime=update diagram  Latency=0  AutoFrameSizeCalculation=off
      link override Signal_Limit/_maxval: Value=KOUTP_V2BDCDCPosRlyFit_enum_maxval
      link override Signal_Limit/_minval: Value=KOUTP_V2BDCDCPosRlyFit_enum_minval
      link override Signal_Override/_ovrdflg: Value=KOUTP_V2BDCDCPosRlyFit_enum_ovrdflg
      link override Signal_Override/_ovrdval: Value=KOUTP_V2BDCDCPosRlyFit_enum_ovrdval
  VPMM_V2BDCDCPosRlySta_enum_Inproc : FVT_lib/outp/OverrideAndLimit  SystemSampleTime=-1  VariantActivationTime=update diagram  Latency=0  AutoFrameSizeCalculation=off
      link override Signal_Limit/_maxval: Value=KOUTP_V2BDCDCPosRlySta_enum_maxval
      link override Signal_Limit/_minval: Value=KOUTP_V2BDCDCPosRlySta_enum_minval
      link override Signal_Override/_ovrdflg: Value=KOUTP_V2BDCDCPosRlySta_enum_ovrdflg
      link override Signal_Override/_ovrdval: Value=KOUTP_V2BDCDCPosRlySta_enum_ovrdval
  VPMM_V2BLifeSig_cnt_Inproc : FVT_lib/outp/OverrideAndLimit  SystemSampleTime=-1  VariantActivationTime=update diagram  Latency=0  AutoFrameSizeCalculation=off
      link override Signal_Limit/_maxval: Value=KOUTP_V2BLifeSig_cnt_maxval
      link override Signal_Limit/_minval: Value=KOUTP_V2BLifeSig_cnt_minval
      link override Signal_Override/_ovrdflg: Value=KOUTP_V2BLifeSig_cnt_ovrdflg
      link override Signal_Override/_ovrdval: Value=KOUTP_V2BLifeSig_cnt_ovrdval
  VPMM_V2BMainPosRlyFit_enum_Inproc : FVT_lib/outp/OverrideAndLimit  SystemSampleTime=-1  VariantActivationTime=update diagram  Latency=0  AutoFrameSizeCalculation=off
      link override Signal_Limit/_maxval: Value=KOUTP_V2BMainPosRlyFit_enum_maxval
      link override Signal_Limit/_minval: Value=KOUTP_V2BMainPosRlyFit_enum_minval
      link override Signal_Override/_ovrdflg: Value=KOUTP_V2BMainPosRlyFit_enum_ovrdflg
      link override Signal_Override/_ovrdval: Value=KOUTP_V2BMainPosRlyFit_enum_ovrdval
  VPMM_V2BMainPosRlySta_enum_Inproc : FVT_lib/outp/OverrideAndLimit  SystemSampleTime=-1  VariantActivationTime=update diagram  Latency=0  AutoFrameSizeCalculation=off
      link override Signal_Limit/_maxval: Value=KOUTP_V2BMainPosRlySta_enum_maxval
      link override Signal_Limit/_minval: Value=KOUTP_V2BMainPosRlySta_enum_minval
      link override Signal_Override/_ovrdflg: Value=KOUTP_V2BMainPosRlySta_enum_ovrdflg
      link override Signal_Override/_ovrdval: Value=KOUTP_V2BMainPosRlySta_enum_ovrdval
  VPMM_V2BOilPosRlyFit_enum_Inproc : FVT_lib/outp/OverrideAndLimit  SystemSampleTime=-1  VariantActivationTime=update diagram  Latency=0  AutoFrameSizeCalculation=off
      link override Signal_Limit/_maxval: Value=KOUTP_V2BOilPosRlyFit_enum_maxval
      link override Signal_Limit/_minval: Value=KOUTP_V2BOilPosRlyFit_enum_minval
      link override Signal_Override/_ovrdflg: Value=KOUTP_V2BOilPosRlyFit_enum_ovrdflg
      link override Signal_Override/_ovrdval: Value=KOUTP_V2BOilPosRlyFit_enum_ovrdval
  VPMM_V2BOilPosRlySta_enum_Inproc : FVT_lib/outp/OverrideAndLimit  SystemSampleTime=-1  VariantActivationTime=update diagram  Latency=0  AutoFrameSizeCalculation=off
      link override Signal_Limit/_maxval: Value=KOUTP_V2BOilPosRlySta_enum_maxval
      link override Signal_Limit/_minval: Value=KOUTP_V2BOilPosRlySta_enum_minval
      link override Signal_Override/_ovrdflg: Value=KOUTP_V2BOilPosRlySta_enum_ovrdflg
      link override Signal_Override/_ovrdval: Value=KOUTP_V2BOilPosRlySta_enum_ovrdval
  VPMM_VCULife1_cnt_Inproc : FVT_lib/outp/OverrideAndLimit  SystemSampleTime=-1  VariantActivationTime=update diagram  Latency=0  AutoFrameSizeCalculation=off
      link override Signal_Limit/_maxval: Value=KOUTP_VCULife1_cnt_maxval
      link override Signal_Limit/_minval: Value=KOUTP_VCULife1_cnt_minval
      link override Signal_Override/_ovrdflg: Value=KOUTP_VCULife1_cnt_ovrdflg
      link override Signal_Override/_ovrdval: Value=KOUTP_VCULife1_cnt_ovrdval
  VPMM_VCULife2_cnt_Inproc : FVT_lib/outp/OverrideAndLimit  SystemSampleTime=-1  VariantActivationTime=update diagram  Latency=0  AutoFrameSizeCalculation=off
      link override Signal_Limit/_maxval: Value=KOUTP_VCULife2_cnt_maxval
      link override Signal_Limit/_minval: Value=KOUTP_VCULife2_cnt_minval
      link override Signal_Override/_ovrdflg: Value=KOUTP_VCULife2_cnt_ovrdflg
      link override Signal_Override/_ovrdval: Value=KOUTP_VCULife2_cnt_ovrdval
  VPMM_VCUMCUEn_flg_Inproc : FVT_lib/outp/OverrideAndLimit  SystemSampleTime=-1  VariantActivationTime=update diagram  Latency=0  AutoFrameSizeCalculation=off
      link override Signal_Limit/_maxval: Value=KOUTP_VCUMCUEn_flg_maxval
      link override Signal_Limit/_minval: Value=KOUTP_VCUMCUEn_flg_minval
      link override Signal_Override/_ovrdflg: Value=KOUTP_VCUMCUEn_flg_ovrdflg
      link override Signal_Override/_ovrdval: Value=KOUTP_VCUMCUEn_flg_ovrdval
  VPMM_VCUMCUFailRst_flg_Inproc : FVT_lib/outp/OverrideAndLimit  SystemSampleTime=-1  VariantActivationTime=update diagram  Latency=0  AutoFrameSizeCalculation=off
      link override Signal_Limit/_maxval: Value=KOUTP_VCUMCUFailRst_flg_maxval
      link override Signal_Limit/_minval: Value=KOUTP_VCUMCUFailRst_flg_minval
      link override Signal_Override/_ovrdflg: Value=KOUTP_VCUMCUFailRst_flg_ovrdflg
      link override Signal_Override/_ovrdval: Value=KOUTP_VCUMCUFailRst_flg_ovrdval
  VPMM_VSPFunc_enum_Inproc : FVT_lib/outp/OverrideAndLimit  SystemSampleTime=-1  VariantActivationTime=update diagram  Latency=0  AutoFrameSizeCalculation=off
      link override Signal_Limit/_maxval: Value=KOUTP_VSPFunc_enum_maxval
      link override Signal_Limit/_minval: Value=KOUTP_VSPFunc_enum_minval
      link override Signal_Override/_ovrdflg: Value=KOUTP_VSPFunc_enum_ovrdflg
      link override Signal_Override/_ovrdval: Value=KOUTP_VSPFunc_enum_ovrdval
  VPMM_VSPIGNKeySta_enum_Inproc : FVT_lib/outp/OverrideAndLimit  SystemSampleTime=-1  VariantActivationTime=update diagram  Latency=0  AutoFrameSizeCalculation=off
      link override Signal_Limit/_maxval: Value=KOUTP_VSPIGNKeySta_enum_maxval
      link override Signal_Limit/_minval: Value=KOUTP_VSPIGNKeySta_enum_minval
      link override Signal_Override/_ovrdflg: Value=KOUTP_VSPIGNKeySta_enum_ovrdflg
      link override Signal_Override/_ovrdval: Value=KOUTP_VSPIGNKeySta_enum_ovrdval
  VPMM_VSPReversed_flg_Inproc : FVT_lib/outp/OverrideAndLimit  SystemSampleTime=-1  VariantActivationTime=update diagram  Latency=0  AutoFrameSizeCalculation=off
      link override Signal_Limit/_maxval: Value=KOUTP_VSPReversed_flg_maxval
      link override Signal_Limit/_minval: Value=KOUTP_VSPReversed_flg_minval
      link override Signal_Override/_ovrdflg: Value=KOUTP_VSPReversed_flg_ovrdflg
      link override Signal_Override/_ovrdval: Value=KOUTP_VSPReversed_flg_ovrdval
  VPMM_VSPTurnLeft_enum_Inproc : FVT_lib/outp/OverrideAndLimit  SystemSampleTime=-1  VariantActivationTime=update diagram  Latency=0  AutoFrameSizeCalculation=off
      link override Signal_Limit/_maxval: Value=KOUTP_VSPTurnLeft_enum_maxval
      link override Signal_Limit/_minval: Value=KOUTP_VSPTurnLeft_enum_minval
      link override Signal_Override/_ovrdflg: Value=KOUTP_VSPTurnLeft_enum_ovrdflg
      link override Signal_Override/_ovrdval: Value=KOUTP_VSPTurnLeft_enum_ovrdval
  VPMM_VSPTurnRight_enum_Inproc : FVT_lib/outp/OverrideAndLimit  SystemSampleTime=-1  VariantActivationTime=update diagram  Latency=0  AutoFrameSizeCalculation=off
      link override Signal_Limit/_maxval: Value=KOUTP_VSPTurnRight_enum_maxval
      link override Signal_Limit/_minval: Value=KOUTP_VSPTurnRight_enum_minval
      link override Signal_Override/_ovrdflg: Value=KOUTP_VSPTurnRight_enum_ovrdflg
      link override Signal_Override/_ovrdval: Value=KOUTP_VSPTurnRight_enum_ovrdval
  VPSA_EmergencyShutDown_flg_Inproc : FVT_lib/outp/OverrideAndLimit  SystemSampleTime=-1  VariantActivationTime=update diagram  Latency=0  AutoFrameSizeCalculation=off
      link override Signal_Limit/_maxval: Value=KOUTP_EmergencyShutDown_flg_maxval
      link override Signal_Limit/_minval: Value=KOUTP_EmergencyShutDown_flg_minval
      link override Signal_Override/_ovrdflg: Value=KOUTP_EmergencyShutDown_flg_ovrdflg
      link override Signal_Override/_ovrdval: Value=KOUTP_EmergencyShutDown_flg_ovrdval
  VPSA_Keystatus_enum_Inproc : FVT_lib/outp/OverrideAndLimit  SystemSampleTime=-1  VariantActivationTime=update diagram  Latency=0  AutoFrameSizeCalculation=off
      link override Signal_Limit/_maxval: Value=KOUTP_Keystatus_enum_maxval
      link override Signal_Limit/_minval: Value=KOUTP_Keystatus_enum_minval
      link override Signal_Override/_ovrdflg: Value=KOUTP_Keystatus_enum_ovrdflg
      link override Signal_Override/_ovrdval: Value=KOUTP_Keystatus_enum_ovrdval
  VSCP_CFGEM1BAMPGN_raw_Inproc : FVT_lib/outp/OverrideAndLimit  SystemSampleTime=-1  VariantActivationTime=update diagram  Latency=0  AutoFrameSizeCalculation=off
      link override Signal_Limit/_maxval: Value=KOUTP_CFGEM1BAMPGN_raw_maxval
      link override Signal_Limit/_minval: Value=KOUTP_CFGEM1BAMPGN_raw_minval
      link override Signal_Override/_ovrdflg: Value=KOUTP_CFGEM1BAMPGN_raw_ovrdflg
      link override Signal_Override/_ovrdval: Value=KOUTP_CFGEM1BAMPGN_raw_ovrdval
  VSCP_CFGEM1BAMRsv_raw_Inproc : FVT_lib/outp/OverrideAndLimit  SystemSampleTime=-1  VariantActivationTime=update diagram  Latency=0  AutoFrameSizeCalculation=off
      link override Signal_Limit/_maxval: Value=KOUTP_CFGEM1BAMRsv_raw_maxval
      link override Signal_Limit/_minval: Value=KOUTP_CFGEM1BAMRsv_raw_minval
      link override Signal_Override/_ovrdflg: Value=KOUTP_CFGEM1BAMRsv_raw_ovrdflg
      link override Signal_Override/_ovrdval: Value=KOUTP_CFGEM1BAMRsv_raw_ovrdval
  VSCP_CFGEM1BAMTNum_raw_Inproc : FVT_lib/outp/OverrideAndLimit  SystemSampleTime=-1  VariantActivationTime=update diagram  Latency=0  AutoFrameSizeCalculation=off
      link override Signal_Limit/_maxval: Value=KOUTP_CFGEM1BAMTNum_raw_maxval
      link override Signal_Limit/_minval: Value=KOUTP_CFGEM1BAMTNum_raw_minval
      link override Signal_Override/_ovrdflg: Value=KOUTP_CFGEM1BAMTNum_raw_ovrdflg
      link override Signal_Override/_ovrdval: Value=KOUTP_CFGEM1BAMTNum_raw_ovrdval
  VSCP_CFGEM1BAMTSize_raw_Inproc : FVT_lib/outp/OverrideAndLimit  SystemSampleTime=-1  VariantActivationTime=update diagram  Latency=0  AutoFrameSizeCalculation=off
      link override Signal_Limit/_maxval: Value=KOUTP_CFGEM1BAMTSize_raw_maxval
      link override Signal_Limit/_minval: Value=KOUTP_CFGEM1BAMTSize_raw_minval
      link override Signal_Override/_ovrdflg: Value=KOUTP_CFGEM1BAMTSize_raw_ovrdflg
      link override Signal_Override/_ovrdval: Value=KOUTP_CFGEM1BAMTSize_raw_ovrdval
  VSCP_CFGEM1Ctrl_raw_Inproc : FVT_lib/outp/OverrideAndLimit  SystemSampleTime=-1  VariantActivationTime=update diagram  Latency=0  AutoFrameSizeCalculation=off
      link override Signal_Limit/_maxval: Value=KOUTP_CFGEM1Ctrl_raw_maxval
      link override Signal_Limit/_minval: Value=KOUTP_CFGEM1Ctrl_raw_minval
      link override Signal_Override/_ovrdflg: Value=KOUTP_CFGEM1Ctrl_raw_ovrdflg
      link override Signal_Override/_ovrdval: Value=KOUTP_CFGEM1Ctrl_raw_ovrdval
  VSCP_DTbyte0_raw_Inproc : FVT_lib/outp/OverrideAndLimit  SystemSampleTime=-1  VariantActivationTime=update diagram  Latency=0  AutoFrameSizeCalculation=off
      link override Signal_Limit/_maxval: Value=KOUTP_DTbyte0_raw_maxval
      link override Signal_Limit/_minval: Value=KOUTP_DTbyte0_raw_minval
      link override Signal_Override/_ovrdflg: Value=KOUTP_DTbyte0_raw_ovrdflg
      link override Signal_Override/_ovrdval: Value=KOUTP_DTbyte0_raw_ovrdval
  VSCP_DTbyte1_raw_Inproc : FVT_lib/outp/OverrideAndLimit  SystemSampleTime=-1  VariantActivationTime=update diagram  Latency=0  AutoFrameSizeCalculation=off
      link override Signal_Limit/_maxval: Value=KOUTP_DTbyte1_raw_maxval
      link override Signal_Limit/_minval: Value=KOUTP_DTbyte1_raw_minval
      link override Signal_Override/_ovrdflg: Value=KOUTP_DTbyte1_raw_ovrdflg
      link override Signal_Override/_ovrdval: Value=KOUTP_DTbyte1_raw_ovrdval
  VSCP_DTbyte2_raw_Inproc : FVT_lib/outp/OverrideAndLimit  SystemSampleTime=-1  VariantActivationTime=update diagram  Latency=0  AutoFrameSizeCalculation=off
      link override Signal_Limit/_maxval: Value=KOUTP_DTbyte2_raw_maxval
      link override Signal_Limit/_minval: Value=KOUTP_DTbyte2_raw_minval
      link override Signal_Override/_ovrdflg: Value=KOUTP_DTbyte2_raw_ovrdflg
      link override Signal_Override/_ovrdval: Value=KOUTP_DTbyte2_raw_ovrdval
  VSCP_DTbyte3_raw_Inproc : FVT_lib/outp/OverrideAndLimit  SystemSampleTime=-1  VariantActivationTime=update diagram  Latency=0  AutoFrameSizeCalculation=off
      link override Signal_Limit/_maxval: Value=KOUTP_DTbyte3_raw_maxval
      link override Signal_Limit/_minval: Value=KOUTP_DTbyte3_raw_minval
      link override Signal_Override/_ovrdflg: Value=KOUTP_DTbyte3_raw_ovrdflg
      link override Signal_Override/_ovrdval: Value=KOUTP_DTbyte3_raw_ovrdval
  VSCP_DTbyte4_raw_Inproc : FVT_lib/outp/OverrideAndLimit  SystemSampleTime=-1  VariantActivationTime=update diagram  Latency=0  AutoFrameSizeCalculation=off
      link override Signal_Limit/_maxval: Value=KOUTP_DTbyte4_raw_maxval
      link override Signal_Limit/_minval: Value=KOUTP_DTbyte4_raw_minval
      link override Signal_Override/_ovrdflg: Value=KOUTP_DTbyte4_raw_ovrdflg
      link override Signal_Override/_ovrdval: Value=KOUTP_DTbyte4_raw_ovrdval
  VSCP_DTbyte5_raw_Inproc : FVT_lib/outp/OverrideAndLimit  SystemSampleTime=-1  VariantActivationTime=update diagram  Latency=0  AutoFrameSizeCalculation=off
      link override Signal_Limit/_maxval: Value=KOUTP_DTbyte5_raw_maxval
      link override Signal_Limit/_minval: Value=KOUTP_DTbyte5_raw_minval
      link override Signal_Override/_ovrdflg: Value=KOUTP_DTbyte5_raw_ovrdflg
      link override Signal_Override/_ovrdval: Value=KOUTP_DTbyte5_raw_ovrdval
  VSCP_DTbyte6_raw_Inproc : FVT_lib/outp/OverrideAndLimit  SystemSampleTime=-1  VariantActivationTime=update diagram  Latency=0  AutoFrameSizeCalculation=off
      link override Signal_Limit/_maxval: Value=KOUTP_DTbyte6_raw_maxval
      link override Signal_Limit/_minval: Value=KOUTP_DTbyte6_raw_minval
      link override Signal_Override/_ovrdflg: Value=KOUTP_DTbyte6_raw_ovrdflg
      link override Signal_Override/_ovrdval: Value=KOUTP_DTbyte6_raw_ovrdval
  VSCP_DTbyte7_raw_Inproc : FVT_lib/outp/OverrideAndLimit  SystemSampleTime=-1  VariantActivationTime=update diagram  Latency=0  AutoFrameSizeCalculation=off
      link override Signal_Limit/_maxval: Value=KOUTP_DTbyte7_raw_maxval
      link override Signal_Limit/_minval: Value=KOUTP_DTbyte7_raw_minval
      link override Signal_Override/_ovrdflg: Value=KOUTP_DTbyte7_raw_ovrdflg
      link override Signal_Override/_ovrdval: Value=KOUTP_DTbyte7_raw_ovrdval
  VSCP_triggerBAM_flg_Inproc : FVT_lib/outp/OverrideAndLimit  SystemSampleTime=-1  VariantActivationTime=update diagram  Latency=0  AutoFrameSizeCalculation=off
      link override Signal_Limit/_maxval: Value=KOUTP_triggerBAM_flg_maxval
      link override Signal_Limit/_minval: Value=KOUTP_triggerBAM_flg_minval
      link override Signal_Override/_ovrdflg: Value=KOUTP_triggerBAM_flg_ovrdflg
      link override Signal_Override/_ovrdval: Value=KOUTP_triggerBAM_flg_ovrdval
  VSCP_triggerDT_flg_Inproc : FVT_lib/outp/OverrideAndLimit  SystemSampleTime=-1  VariantActivationTime=update diagram  Latency=0  AutoFrameSizeCalculation=off
      link override Signal_Limit/_maxval: Value=KOUTP_triggerDT_flg_maxval
      link override Signal_Limit/_minval: Value=KOUTP_triggerDT_flg_minval
      link override Signal_Override/_ovrdflg: Value=KOUTP_triggerDT_flg_ovrdflg
      link override Signal_Override/_ovrdval: Value=KOUTP_triggerDT_flg_ovrdval
  VSYS_AcoreRebootCmdACK_flg_Inproc : FVT_lib/outp/OverrideAndLimit  SystemSampleTime=-1  VariantActivationTime=update diagram  Latency=0  AutoFrameSizeCalculation=off
      link override Signal_Limit/_maxval: Value=KOUTP_AcoreRebootCmdACK_flg_maxval
      link override Signal_Limit/_minval: Value=KOUTP_AcoreRebootCmdACK_flg_minval
      link override Signal_Override/_ovrdflg: Value=KOUTP_AcoreRebootCmdACK_flg_ovrdflg
      link override Signal_Override/_ovrdval: Value=KOUTP_AcoreRebootCmdACK_flg_ovrdval
  VSYS_CarModel1_cnt_Inproc : FVT_lib/outp/OverrideAndLimit  SystemSampleTime=-1  VariantActivationTime=update diagram  Latency=0  AutoFrameSizeCalculation=off
      link override Signal_Limit/_maxval: Value=KOUTP_CarModel1_cnt_maxval
      link override Signal_Limit/_minval: Value=KOUTP_CarModel1_cnt_minval
      link override Signal_Override/_ovrdflg: Value=KOUTP_CarModel1_cnt_ovrdflg
      link override Signal_Override/_ovrdval: Value=KOUTP_CarModel1_cnt_ovrdval
  VSYS_CarModel2_cnt_Inproc : FVT_lib/outp/OverrideAndLimit  SystemSampleTime=-1  VariantActivationTime=update diagram  Latency=0  AutoFrameSizeCalculation=off
      link override Signal_Limit/_maxval: Value=KOUTP_CarModel2_cnt_maxval
      link override Signal_Limit/_minval: Value=KOUTP_CarModel2_cnt_minval
      link override Signal_Override/_ovrdflg: Value=KOUTP_CarModel2_cnt_ovrdflg
      link override Signal_Override/_ovrdval: Value=KOUTP_CarModel2_cnt_ovrdval
  VSYS_CarModel3_cnt_Inproc : FVT_lib/outp/OverrideAndLimit  SystemSampleTime=-1  VariantActivationTime=update diagram  Latency=0  AutoFrameSizeCalculation=off
      link override Signal_Limit/_maxval: Value=KOUTP_CarModel3_cnt_maxval
      link override Signal_Limit/_minval: Value=KOUTP_CarModel3_cnt_minval
      link override Signal_Override/_ovrdflg: Value=KOUTP_CarModel3_cnt_ovrdflg
      link override Signal_Override/_ovrdval: Value=KOUTP_CarModel3_cnt_ovrdval
  VSYS_Change1_cnt_Inproc : FVT_lib/outp/OverrideAndLimit  SystemSampleTime=-1  VariantActivationTime=update diagram  Latency=0  AutoFrameSizeCalculation=off
      link override Signal_Limit/_maxval: Value=KOUTP_Change1_cnt_maxval
      link override Signal_Limit/_minval: Value=KOUTP_Change1_cnt_minval
      link override Signal_Override/_ovrdflg: Value=KOUTP_Change1_cnt_ovrdflg
      link override Signal_Override/_ovrdval: Value=KOUTP_Change1_cnt_ovrdval
  VSYS_Change2_cnt_Inproc : FVT_lib/outp/OverrideAndLimit  SystemSampleTime=-1  VariantActivationTime=update diagram  Latency=0  AutoFrameSizeCalculation=off
      link override Signal_Limit/_maxval: Value=KOUTP_Change2_cnt_maxval
      link override Signal_Limit/_minval: Value=KOUTP_Change2_cnt_minval
      link override Signal_Override/_ovrdflg: Value=KOUTP_Change2_cnt_ovrdflg
      link override Signal_Override/_ovrdval: Value=KOUTP_Change2_cnt_ovrdval
  VSYS_Country1_cnt_Inproc : FVT_lib/outp/OverrideAndLimit  SystemSampleTime=-1  VariantActivationTime=update diagram  Latency=0  AutoFrameSizeCalculation=off
      link override Signal_Limit/_maxval: Value=KOUTP_Country1_cnt_maxval
      link override Signal_Limit/_minval: Value=KOUTP_Country1_cnt_minval
      link override Signal_Override/_ovrdflg: Value=KOUTP_Country1_cnt_ovrdflg
      link override Signal_Override/_ovrdval: Value=KOUTP_Country1_cnt_ovrdval
  VSYS_Country2_cnt_Inproc : FVT_lib/outp/OverrideAndLimit  SystemSampleTime=-1  VariantActivationTime=update diagram  Latency=0  AutoFrameSizeCalculation=off
      link override Signal_Limit/_maxval: Value=KOUTP_Country2_cnt_maxval
      link override Signal_Limit/_minval: Value=KOUTP_Country2_cnt_minval
      link override Signal_Override/_ovrdflg: Value=KOUTP_Country2_cnt_ovrdflg
      link override Signal_Override/_ovrdval: Value=KOUTP_Country2_cnt_ovrdval
  VSYS_CurrentNmState_enum_Inproc : FVT_lib/outp/OverrideAndLimit  SystemSampleTime=-1  VariantActivationTime=update diagram  Latency=0  AutoFrameSizeCalculation=off
      link override Signal_Limit/_maxval: Value=KOUTP_CurrentNmState_enum_maxval
      link override Signal_Limit/_minval: Value=KOUTP_CurrentNmState_enum_minval
      link override Signal_Override/_ovrdflg: Value=KOUTP_CurrentNmState_enum_ovrdflg
      link override Signal_Override/_ovrdval: Value=KOUTP_CurrentNmState_enum_ovrdval
  VSYS_Dash1_cnt_Inproc : FVT_lib/outp/OverrideAndLimit  SystemSampleTime=-1  VariantActivationTime=update diagram  Latency=0  AutoFrameSizeCalculation=off
      link override Signal_Limit/_maxval: Value=KOUTP_Dash1_cnt_maxval
      link override Signal_Limit/_minval: Value=KOUTP_Dash1_cnt_minval
      link override Signal_Override/_ovrdflg: Value=KOUTP_Dash1_cnt_ovrdflg
      link override Signal_Override/_ovrdval: Value=KOUTP_Dash1_cnt_ovrdval
  VSYS_Dash2_cnt_Inproc : FVT_lib/outp/OverrideAndLimit  SystemSampleTime=-1  VariantActivationTime=update diagram  Latency=0  AutoFrameSizeCalculation=off
      link override Signal_Limit/_maxval: Value=KOUTP_Dash2_cnt_maxval
      link override Signal_Limit/_minval: Value=KOUTP_Dash2_cnt_minval
      link override Signal_Override/_ovrdflg: Value=KOUTP_Dash2_cnt_ovrdflg
      link override Signal_Override/_ovrdval: Value=KOUTP_Dash2_cnt_ovrdval
  VSYS_DrivingMode_cnt_Inproc : FVT_lib/outp/OverrideAndLimit  SystemSampleTime=-1  VariantActivationTime=update diagram  Latency=0  AutoFrameSizeCalculation=off
      link override Signal_Limit/_maxval: Value=KOUTP_DrivingMode_cnt_maxval
      link override Signal_Limit/_minval: Value=KOUTP_DrivingMode_cnt_minval
      link override Signal_Override/_ovrdflg: Value=KOUTP_DrivingMode_cnt_ovrdflg
      link override Signal_Override/_ovrdval: Value=KOUTP_DrivingMode_cnt_ovrdval
  VSYS_ECU1_cnt_Inproc : FVT_lib/outp/OverrideAndLimit  SystemSampleTime=-1  VariantActivationTime=update diagram  Latency=0  AutoFrameSizeCalculation=off
      link override Signal_Limit/_maxval: Value=KOUTP_ECU1_cnt_maxval
      link override Signal_Limit/_minval: Value=KOUTP_ECU1_cnt_minval
      link override Signal_Override/_ovrdflg: Value=KOUTP_ECU1_cnt_ovrdflg
      link override Signal_Override/_ovrdval: Value=KOUTP_ECU1_cnt_ovrdval
  VSYS_ECU2_cnt_Inproc : FVT_lib/outp/OverrideAndLimit  SystemSampleTime=-1  VariantActivationTime=update diagram  Latency=0  AutoFrameSizeCalculation=off
      link override Signal_Limit/_maxval: Value=KOUTP_ECU2_cnt_maxval
      link override Signal_Limit/_minval: Value=KOUTP_ECU2_cnt_minval
      link override Signal_Override/_ovrdflg: Value=KOUTP_ECU2_cnt_ovrdflg
      link override Signal_Override/_ovrdval: Value=KOUTP_ECU2_cnt_ovrdval
  VSYS_ECUGen1_cnt_Inproc : FVT_lib/outp/OverrideAndLimit  SystemSampleTime=-1  VariantActivationTime=update diagram  Latency=0  AutoFrameSizeCalculation=off
      link override Signal_Limit/_maxval: Value=KOUTP_ECUGen1_cnt_maxval
      link override Signal_Limit/_minval: Value=KOUTP_ECUGen1_cnt_minval
      link override Signal_Override/_ovrdflg: Value=KOUTP_ECUGen1_cnt_ovrdflg
      link override Signal_Override/_ovrdval: Value=KOUTP_ECUGen1_cnt_ovrdval
  VSYS_ECUGen2_cnt_Inproc : FVT_lib/outp/OverrideAndLimit  SystemSampleTime=-1  VariantActivationTime=update diagram  Latency=0  AutoFrameSizeCalculation=off
      link override Signal_Limit/_maxval: Value=KOUTP_ECUGen2_cnt_maxval
      link override Signal_Limit/_minval: Value=KOUTP_ECUGen2_cnt_minval
      link override Signal_Override/_ovrdflg: Value=KOUTP_ECUGen2_cnt_ovrdflg
      link override Signal_Override/_ovrdval: Value=KOUTP_ECUGen2_cnt_ovrdval
  VSYS_FdcSlpReqRisingEdge_flg_Inproc : FVT_lib/outp/OverrideAndLimit  SystemSampleTime=-1  VariantActivationTime=update diagram  Latency=0  AutoFrameSizeCalculation=off
      link override Signal_Limit/_maxval: Value=KOUTP_FdcSlpReqRisingEdge_flg_maxval
      link override Signal_Limit/_minval: Value=KOUTP_FdcSlpReqRisingEdge_flg_minval
      link override Signal_Override/_ovrdflg: Value=KOUTP_FdcSlpReqRisingEdge_flg_ovrdflg
      link override Signal_Override/_ovrdval: Value=KOUTP_FdcSlpReqRisingEdge_flg_ovrdval
  VSYS_FdcSlpTime_sec_Inproc : FVT_lib/outp/OverrideAndLimit  SystemSampleTime=-1  VariantActivationTime=update diagram  Latency=0  AutoFrameSizeCalculation=off
      link override Signal_Limit/_maxval: Value=KOUTP_FdcSlpTime_sec_maxval
      link override Signal_Limit/_minval: Value=KOUTP_FdcSlpTime_sec_minval
      link override Signal_Override/_ovrdflg: Value=KOUTP_FdcSlpTime_sec_ovrdflg
      link override Signal_Override/_ovrdval: Value=KOUTP_FdcSlpTime_sec_ovrdval
  VSYS_HWVer1_cnt_Inproc : FVT_lib/outp/OverrideAndLimit  SystemSampleTime=-1  VariantActivationTime=update diagram  Latency=0  AutoFrameSizeCalculation=off
      link override Signal_Limit/_maxval: Value=KOUTP_HWVer1_cnt_maxval
      link override Signal_Limit/_minval: Value=KOUTP_HWVer1_cnt_minval
      link override Signal_Override/_ovrdflg: Value=KOUTP_HWVer1_cnt_ovrdflg
      link override Signal_Override/_ovrdval: Value=KOUTP_HWVer1_cnt_ovrdval
  VSYS_HWVer2_cnt_Inproc : FVT_lib/outp/OverrideAndLimit  SystemSampleTime=-1  VariantActivationTime=update diagram  Latency=0  AutoFrameSizeCalculation=off
      link override Signal_Limit/_maxval: Value=KOUTP_HWVer2_cnt_maxval
      link override Signal_Limit/_minval: Value=KOUTP_HWVer2_cnt_minval
      link override Signal_Override/_ovrdflg: Value=KOUTP_HWVer2_cnt_ovrdflg
      link override Signal_Override/_ovrdval: Value=KOUTP_HWVer2_cnt_ovrdval
  VSYS_HWVer3_cnt_Inproc : FVT_lib/outp/OverrideAndLimit  SystemSampleTime=-1  VariantActivationTime=update diagram  Latency=0  AutoFrameSizeCalculation=off
      link override Signal_Limit/_maxval: Value=KOUTP_HWVer3_cnt_maxval
      link override Signal_Limit/_minval: Value=KOUTP_HWVer3_cnt_minval
      link override Signal_Override/_ovrdflg: Value=KOUTP_HWVer3_cnt_ovrdflg
      link override Signal_Override/_ovrdval: Value=KOUTP_HWVer3_cnt_ovrdval
  VSYS_Major1_cnt_Inproc : FVT_lib/outp/OverrideAndLimit  SystemSampleTime=-1  VariantActivationTime=update diagram  Latency=0  AutoFrameSizeCalculation=off
      link override Signal_Limit/_maxval: Value=KOUTP_Major1_cnt_maxval
      link override Signal_Limit/_minval: Value=KOUTP_Major1_cnt_minval
      link override Signal_Override/_ovrdflg: Value=KOUTP_Major1_cnt_ovrdflg
      link override Signal_Override/_ovrdval: Value=KOUTP_Major1_cnt_ovrdval
  VSYS_Major2_cnt_Inproc : FVT_lib/outp/OverrideAndLimit  SystemSampleTime=-1  VariantActivationTime=update diagram  Latency=0  AutoFrameSizeCalculation=off
      link override Signal_Limit/_maxval: Value=KOUTP_Major2_cnt_maxval
      link override Signal_Limit/_minval: Value=KOUTP_Major2_cnt_minval
      link override Signal_Override/_ovrdflg: Value=KOUTP_Major2_cnt_ovrdflg
      link override Signal_Override/_ovrdval: Value=KOUTP_Major2_cnt_ovrdval
  VSYS_Minor1_cnt_Inproc : FVT_lib/outp/OverrideAndLimit  SystemSampleTime=-1  VariantActivationTime=update diagram  Latency=0  AutoFrameSizeCalculation=off
      link override Signal_Limit/_maxval: Value=KOUTP_Minor1_cnt_maxval
      link override Signal_Limit/_minval: Value=KOUTP_Minor1_cnt_minval
      link override Signal_Override/_ovrdflg: Value=KOUTP_Minor1_cnt_ovrdflg
      link override Signal_Override/_ovrdval: Value=KOUTP_Minor1_cnt_ovrdval
  VSYS_Minor2_cnt_Inproc : FVT_lib/outp/OverrideAndLimit  SystemSampleTime=-1  VariantActivationTime=update diagram  Latency=0  AutoFrameSizeCalculation=off
      link override Signal_Limit/_maxval: Value=KOUTP_Minor2_cnt_maxval
      link override Signal_Limit/_minval: Value=KOUTP_Minor2_cnt_minval
      link override Signal_Override/_ovrdflg: Value=KOUTP_Minor2_cnt_ovrdflg
      link override Signal_Override/_ovrdval: Value=KOUTP_Minor2_cnt_ovrdval
  VSYS_ModelYear_cnt_Inproc : FVT_lib/outp/OverrideAndLimit  SystemSampleTime=-1  VariantActivationTime=update diagram  Latency=0  AutoFrameSizeCalculation=off
      link override Signal_Limit/_maxval: Value=KOUTP_ModelYear_cnt_maxval
      link override Signal_Limit/_minval: Value=KOUTP_ModelYear_cnt_minval
      link override Signal_Override/_ovrdflg: Value=KOUTP_ModelYear_cnt_ovrdflg
      link override Signal_Override/_ovrdval: Value=KOUTP_ModelYear_cnt_ovrdval
  VSYS_NvWriteReqRisingEdge_flg_Inproc : FVT_lib/outp/OverrideAndLimit  SystemSampleTime=-1  VariantActivationTime=update diagram  Latency=0  AutoFrameSizeCalculation=off
      link override Signal_Limit/_maxval: Value=KOUTP_NvWriteReqRisingEdge_flg_maxval
      link override Signal_Limit/_minval: Value=KOUTP_NvWriteReqRisingEdge_flg_minval
      link override Signal_Override/_ovrdflg: Value=KOUTP_NvWriteReqRisingEdge_flg_ovrdflg
      link override Signal_Override/_ovrdval: Value=KOUTP_NvWriteReqRisingEdge_flg_ovrdval
  VSYS_Patch1_cnt_Inproc : FVT_lib/outp/OverrideAndLimit  SystemSampleTime=-1  VariantActivationTime=update diagram  Latency=0  AutoFrameSizeCalculation=off
      link override Signal_Limit/_maxval: Value=KOUTP_Patch1_cnt_maxval
      link override Signal_Limit/_minval: Value=KOUTP_Patch1_cnt_minval
      link override Signal_Override/_ovrdflg: Value=KOUTP_Patch1_cnt_ovrdflg
      link override Signal_Override/_ovrdval: Value=KOUTP_Patch1_cnt_ovrdval
  VSYS_Patch2_cnt_Inproc : FVT_lib/outp/OverrideAndLimit  SystemSampleTime=-1  VariantActivationTime=update diagram  Latency=0  AutoFrameSizeCalculation=off
      link override Signal_Limit/_maxval: Value=KOUTP_Patch2_cnt_maxval
      link override Signal_Limit/_minval: Value=KOUTP_Patch2_cnt_minval
      link override Signal_Override/_ovrdflg: Value=KOUTP_Patch2_cnt_ovrdflg
      link override Signal_Override/_ovrdval: Value=KOUTP_Patch2_cnt_ovrdval
  VSYS_PmicBootPath_raw32_Inproc : FVT_lib/outp/OverrideAndLimit  SystemSampleTime=-1  VariantActivationTime=update diagram  Latency=0  AutoFrameSizeCalculation=off
      link override Signal_Limit/_maxval: Value=KOUTP_PmicBootPath_raw32_maxval
      link override Signal_Limit/_minval: Value=KOUTP_PmicBootPath_raw32_minval
      link override Signal_Override/_ovrdflg: Value=KOUTP_PmicBootPath_raw32_ovrdflg
      link override Signal_Override/_ovrdval: Value=KOUTP_PmicBootPath_raw32_ovrdval
  VSYS_PmicBootReason_enum_Inproc : FVT_lib/outp/OverrideAndLimit  SystemSampleTime=-1  VariantActivationTime=update diagram  Latency=0  AutoFrameSizeCalculation=off
      link override Signal_Limit/_maxval: Value=KOUTP_PmicBootReason_enum_maxval
      link override Signal_Limit/_minval: Value=KOUTP_PmicBootReason_enum_minval
      link override Signal_Override/_ovrdflg: Value=KOUTP_PmicBootReason_enum_ovrdflg
      link override Signal_Override/_ovrdval: Value=KOUTP_PmicBootReason_enum_ovrdval
  VSYS_SHA1_cnt_Inproc : FVT_lib/outp/OverrideAndLimit  SystemSampleTime=-1  VariantActivationTime=update diagram  Latency=0  AutoFrameSizeCalculation=off
      link override Signal_Limit/_maxval: Value=KOUTP_SHA1_cnt_maxval
      link override Signal_Limit/_minval: Value=KOUTP_SHA1_cnt_minval
      link override Signal_Override/_ovrdflg: Value=KOUTP_SHA1_cnt_ovrdflg
      link override Signal_Override/_ovrdval: Value=KOUTP_SHA1_cnt_ovrdval
  VSYS_SHA2_cnt_Inproc : FVT_lib/outp/OverrideAndLimit  SystemSampleTime=-1  VariantActivationTime=update diagram  Latency=0  AutoFrameSizeCalculation=off
      link override Signal_Limit/_maxval: Value=KOUTP_SHA2_cnt_maxval
      link override Signal_Limit/_minval: Value=KOUTP_SHA2_cnt_minval
      link override Signal_Override/_ovrdflg: Value=KOUTP_SHA2_cnt_ovrdflg
      link override Signal_Override/_ovrdval: Value=KOUTP_SHA2_cnt_ovrdval
  VSYS_SHA3_cnt_Inproc : FVT_lib/outp/OverrideAndLimit  SystemSampleTime=-1  VariantActivationTime=update diagram  Latency=0  AutoFrameSizeCalculation=off
      link override Signal_Limit/_maxval: Value=KOUTP_SHA3_cnt_maxval
      link override Signal_Limit/_minval: Value=KOUTP_SHA3_cnt_minval
      link override Signal_Override/_ovrdflg: Value=KOUTP_SHA3_cnt_ovrdflg
      link override Signal_Override/_ovrdval: Value=KOUTP_SHA3_cnt_ovrdval
  VSYS_SHA4_cnt_Inproc : FVT_lib/outp/OverrideAndLimit  SystemSampleTime=-1  VariantActivationTime=update diagram  Latency=0  AutoFrameSizeCalculation=off
      link override Signal_Limit/_maxval: Value=KOUTP_SHA4_cnt_maxval
      link override Signal_Limit/_minval: Value=KOUTP_SHA4_cnt_minval
      link override Signal_Override/_ovrdflg: Value=KOUTP_SHA4_cnt_ovrdflg
      link override Signal_Override/_ovrdval: Value=KOUTP_SHA4_cnt_ovrdval
  VSYS_SHA5_cnt_Inproc : FVT_lib/outp/OverrideAndLimit  SystemSampleTime=-1  VariantActivationTime=update diagram  Latency=0  AutoFrameSizeCalculation=off
      link override Signal_Limit/_maxval: Value=KOUTP_SHA5_cnt_maxval
      link override Signal_Limit/_minval: Value=KOUTP_SHA5_cnt_minval
      link override Signal_Override/_ovrdflg: Value=KOUTP_SHA5_cnt_ovrdflg
      link override Signal_Override/_ovrdval: Value=KOUTP_SHA5_cnt_ovrdval
  VSYS_SHA6_cnt_Inproc : FVT_lib/outp/OverrideAndLimit  SystemSampleTime=-1  VariantActivationTime=update diagram  Latency=0  AutoFrameSizeCalculation=off
      link override Signal_Limit/_maxval: Value=KOUTP_SHA6_cnt_maxval
      link override Signal_Limit/_minval: Value=KOUTP_SHA6_cnt_minval
      link override Signal_Override/_ovrdflg: Value=KOUTP_SHA6_cnt_ovrdflg
      link override Signal_Override/_ovrdval: Value=KOUTP_SHA6_cnt_ovrdval
  VSYS_SHA7_cnt_Inproc : FVT_lib/outp/OverrideAndLimit  SystemSampleTime=-1  VariantActivationTime=update diagram  Latency=0  AutoFrameSizeCalculation=off
      link override Signal_Limit/_maxval: Value=KOUTP_SHA7_cnt_maxval
      link override Signal_Limit/_minval: Value=KOUTP_SHA7_cnt_minval
      link override Signal_Override/_ovrdflg: Value=KOUTP_SHA7_cnt_ovrdflg
      link override Signal_Override/_ovrdval: Value=KOUTP_SHA7_cnt_ovrdval
  VSYS_SHA8_cnt_Inproc : FVT_lib/outp/OverrideAndLimit  SystemSampleTime=-1  VariantActivationTime=update diagram  Latency=0  AutoFrameSizeCalculation=off
      link override Signal_Limit/_maxval: Value=KOUTP_SHA8_cnt_maxval
      link override Signal_Limit/_minval: Value=KOUTP_SHA8_cnt_minval
      link override Signal_Override/_ovrdflg: Value=KOUTP_SHA8_cnt_ovrdflg
      link override Signal_Override/_ovrdval: Value=KOUTP_SHA8_cnt_ovrdval
  VSYS_Variation_cnt_Inproc : FVT_lib/outp/OverrideAndLimit  SystemSampleTime=-1  VariantActivationTime=update diagram  Latency=0  AutoFrameSizeCalculation=off
      link override Signal_Limit/_maxval: Value=KOUTP_Variation_cnt_maxval
      link override Signal_Limit/_minval: Value=KOUTP_Variation_cnt_minval
      link override Signal_Override/_ovrdflg: Value=KOUTP_Variation_cnt_ovrdflg
      link override Signal_Override/_ovrdval: Value=KOUTP_Variation_cnt_ovrdval
  VSYS_WisrBootReason_raw32_Inproc : FVT_lib/outp/OverrideAndLimit  SystemSampleTime=-1  VariantActivationTime=update diagram  Latency=0  AutoFrameSizeCalculation=off
      link override Signal_Limit/_maxval: Value=KOUTP_WisrBootReason_raw32_maxval
      link override Signal_Limit/_minval: Value=KOUTP_WisrBootReason_raw32_minval
      link override Signal_Override/_ovrdflg: Value=KOUTP_WisrBootReason_raw32_ovrdflg
      link override Signal_Override/_ovrdval: Value=KOUTP_WisrBootReason_raw32_ovrdval
  VTHC_AfterrunningMode_flg_Inproc : FVT_lib/outp/OverrideAndLimit  SystemSampleTime=-1  VariantActivationTime=update diagram  Latency=0  AutoFrameSizeCalculation=off
      link override Signal_Limit/_maxval: Value=KOUTP_AfterrunningMode_flg_maxval
      link override Signal_Limit/_minval: Value=KOUTP_AfterrunningMode_flg_minval
      link override Signal_Override/_ovrdflg: Value=KOUTP_AfterrunningMode_flg_ovrdflg
      link override Signal_Override/_ovrdval: Value=KOUTP_AfterrunningMode_flg_ovrdval
  VTHC_CoolFanReq_pct_Inproc : FVT_lib/outp/OverrideAndLimit  SystemSampleTime=-1  VariantActivationTime=update diagram  Latency=0  AutoFrameSizeCalculation=off
      link override Signal_Limit/_maxval: Value=KOUTP_CoolFanReq_pct_maxval
      link override Signal_Limit/_minval: Value=KOUTP_CoolFanReq_pct_minval
      link override Signal_Override/_ovrdflg: Value=KOUTP_CoolFanReq_pct_ovrdflg
      link override Signal_Override/_ovrdval: Value=KOUTP_CoolFanReq_pct_ovrdval
  VTHC_EWPPEReq_rpm_Inproc : FVT_lib/outp/OverrideAndLimit  SystemSampleTime=-1  VariantActivationTime=update diagram  Latency=0  AutoFrameSizeCalculation=off
      link override Signal_Limit/_maxval: Value=KOUTP_EWPPEReq_rpm_maxval
      link override Signal_Limit/_minval: Value=KOUTP_EWPPEReq_rpm_minval
      link override Signal_Override/_ovrdflg: Value=KOUTP_EWPPEReq_rpm_ovrdflg
      link override Signal_Override/_ovrdval: Value=KOUTP_EWPPEReq_rpm_ovrdval
  VTPM_ALFin_flg_Inproc : FVT_lib/outp/OverrideAndLimit  SystemSampleTime=-1  VariantActivationTime=update diagram  Latency=0  AutoFrameSizeCalculation=off
      link override Signal_Limit/_maxval: Value=KOUTP_ALFin_flg_maxval
      link override Signal_Limit/_minval: Value=KOUTP_ALFin_flg_minval
      link override Signal_Override/_ovrdflg: Value=KOUTP_ALFin_flg_ovrdflg
      link override Signal_Override/_ovrdval: Value=KOUTP_ALFin_flg_ovrdval
  VTPM_AutoLTips_enum_Inproc : FVT_lib/outp/OverrideAndLimit  SystemSampleTime=-1  VariantActivationTime=update diagram  Latency=0  AutoFrameSizeCalculation=off
      link override Signal_Limit/_maxval: Value=KOUTP_AutoLTips_enum_maxval
      link override Signal_Limit/_minval: Value=KOUTP_AutoLTips_enum_minval
      link override Signal_Override/_ovrdflg: Value=KOUTP_AutoLTips_enum_ovrdflg
      link override Signal_Override/_ovrdval: Value=KOUTP_AutoLTips_enum_ovrdval
  VTPM_CWheelTips_enum_Inproc : FVT_lib/outp/OverrideAndLimit  SystemSampleTime=-1  VariantActivationTime=update diagram  Latency=0  AutoFrameSizeCalculation=off
      link override Signal_Limit/_maxval: Value=KOUTP_CWheelTips_enum_maxval
      link override Signal_Limit/_minval: Value=KOUTP_CWheelTips_enum_minval
      link override Signal_Override/_ovrdflg: Value=KOUTP_CWheelTips_enum_ovrdflg
      link override Signal_Override/_ovrdval: Value=KOUTP_CWheelTips_enum_ovrdval
  VTPM_ChkStorge_flg_Inproc : FVT_lib/outp/OverrideAndLimit  SystemSampleTime=-1  VariantActivationTime=update diagram  Latency=0  AutoFrameSizeCalculation=off
      link override Signal_Limit/_maxval: Value=KOUTP_ChkStorge_flg_maxval
      link override Signal_Limit/_minval: Value=KOUTP_ChkStorge_flg_minval
      link override Signal_Override/_ovrdflg: Value=KOUTP_ChkStorge_flg_ovrdflg
      link override Signal_Override/_ovrdval: Value=KOUTP_ChkStorge_flg_ovrdval
  VTPM_Chkfin_flg_Inproc : FVT_lib/outp/OverrideAndLimit  SystemSampleTime=-1  VariantActivationTime=update diagram  Latency=0  AutoFrameSizeCalculation=off
      link override Signal_Limit/_maxval: Value=KOUTP_Chkfin_flg_maxval
      link override Signal_Limit/_minval: Value=KOUTP_Chkfin_flg_minval
      link override Signal_Override/_ovrdflg: Value=KOUTP_Chkfin_flg_ovrdflg
      link override Signal_Override/_ovrdval: Value=KOUTP_Chkfin_flg_ovrdval
  VTPM_FAT_flg_Inproc : FVT_lib/outp/OverrideAndLimit  SystemSampleTime=-1  VariantActivationTime=update diagram  Latency=0  AutoFrameSizeCalculation=off
      link override Signal_Limit/_maxval: Value=KOUTP_FAT_flg_maxval
      link override Signal_Limit/_minval: Value=KOUTP_FAT_flg_minval
      link override Signal_Override/_ovrdflg: Value=KOUTP_FAT_flg_ovrdflg
      link override Signal_Override/_ovrdval: Value=KOUTP_FAT_flg_ovrdval
  VTPM_FlashIDvalid_enum_Inproc : FVT_lib/outp/OverrideAndLimit  SystemSampleTime=-1  VariantActivationTime=update diagram  Latency=0  AutoFrameSizeCalculation=off
      link override Signal_Limit/_maxval: Value=KOUTP_FlashIDvalid_enum_maxval
      link override Signal_Limit/_minval: Value=KOUTP_FlashIDvalid_enum_minval
      link override Signal_Override/_ovrdflg: Value=KOUTP_FlashIDvalid_enum_ovrdflg
      link override Signal_Override/_ovrdval: Value=KOUTP_FlashIDvalid_enum_ovrdval
  VTPM_FlashS1ID_raw_Inproc : FVT_lib/outp/OverrideAndLimit  SystemSampleTime=-1  VariantActivationTime=update diagram  Latency=0  AutoFrameSizeCalculation=off
      link override Signal_Limit/_maxval: Value=KOUTP_FlashS1ID_raw_maxval
      link override Signal_Limit/_minval: Value=KOUTP_FlashS1ID_raw_minval
      link override Signal_Override/_ovrdflg: Value=KOUTP_FlashS1ID_raw_ovrdflg
      link override Signal_Override/_ovrdval: Value=KOUTP_FlashS1ID_raw_ovrdval
  VTPM_FlashS2ID_raw_Inproc : FVT_lib/outp/OverrideAndLimit  SystemSampleTime=-1  VariantActivationTime=update diagram  Latency=0  AutoFrameSizeCalculation=off
      link override Signal_Limit/_maxval: Value=KOUTP_FlashS2ID_raw_maxval
      link override Signal_Limit/_minval: Value=KOUTP_FlashS2ID_raw_minval
      link override Signal_Override/_ovrdflg: Value=KOUTP_FlashS2ID_raw_ovrdflg
      link override Signal_Override/_ovrdval: Value=KOUTP_FlashS2ID_raw_ovrdval
  VTPM_FlashS3ID_raw_Inproc : FVT_lib/outp/OverrideAndLimit  SystemSampleTime=-1  VariantActivationTime=update diagram  Latency=0  AutoFrameSizeCalculation=off
      link override Signal_Limit/_maxval: Value=KOUTP_FlashS3ID_raw_maxval
      link override Signal_Limit/_minval: Value=KOUTP_FlashS3ID_raw_minval
      link override Signal_Override/_ovrdflg: Value=KOUTP_FlashS3ID_raw_ovrdflg
      link override Signal_Override/_ovrdval: Value=KOUTP_FlashS3ID_raw_ovrdval
  VTPM_FlashS4ID_raw_Inproc : FVT_lib/outp/OverrideAndLimit  SystemSampleTime=-1  VariantActivationTime=update diagram  Latency=0  AutoFrameSizeCalculation=off
      link override Signal_Limit/_maxval: Value=KOUTP_FlashS4ID_raw_maxval
      link override Signal_Limit/_minval: Value=KOUTP_FlashS4ID_raw_minval
      link override Signal_Override/_ovrdflg: Value=KOUTP_FlashS4ID_raw_ovrdflg
      link override Signal_Override/_ovrdval: Value=KOUTP_FlashS4ID_raw_ovrdval
  VTPM_Flashchkdatavalid_enum_Inproc : FVT_lib/outp/OverrideAndLimit  SystemSampleTime=-1  VariantActivationTime=update diagram  Latency=0  AutoFrameSizeCalculation=off
      link override Signal_Limit/_maxval: Value=KOUTP_Flashchkdatavalid_enum_maxval
      link override Signal_Limit/_minval: Value=KOUTP_Flashchkdatavalid_enum_minval
      link override Signal_Override/_ovrdflg: Value=KOUTP_Flashchkdatavalid_enum_ovrdflg
      link override Signal_Override/_ovrdval: Value=KOUTP_Flashchkdatavalid_enum_ovrdval
  VTPM_Flashdatavalid_enum_Inproc : FVT_lib/outp/OverrideAndLimit  SystemSampleTime=-1  VariantActivationTime=update diagram  Latency=0  AutoFrameSizeCalculation=off
      link override Signal_Limit/_maxval: Value=KOUTP_Flashdatavalid_enum_maxval
      link override Signal_Limit/_minval: Value=KOUTP_Flashdatavalid_enum_minval
      link override Signal_Override/_ovrdflg: Value=KOUTP_Flashdatavalid_enum_ovrdflg
      link override Signal_Override/_ovrdval: Value=KOUTP_Flashdatavalid_enum_ovrdval
  VTPM_ID1messageALTU_raw8_Inproc : FVT_lib/outp/OverrideAndLimit  SystemSampleTime=-1  VariantActivationTime=update diagram  Latency=0  AutoFrameSizeCalculation=off
      link override Signal_Limit/_maxval: Value=KOUTP_ID1messageALTU_raw8_maxval
      link override Signal_Limit/_minval: Value=KOUTP_ID1messageALTU_raw8_minval
      link override Signal_Override/_ovrdflg: Value=KOUTP_ID1messageALTU_raw8_ovrdflg
      link override Signal_Override/_ovrdval: Value=KOUTP_ID1messageALTU_raw8_ovrdval
  VTPM_ID2messageALTU_raw8_Inproc : FVT_lib/outp/OverrideAndLimit  SystemSampleTime=-1  VariantActivationTime=update diagram  Latency=0  AutoFrameSizeCalculation=off
      link override Signal_Limit/_maxval: Value=KOUTP_ID2messageALTU_raw8_maxval
      link override Signal_Limit/_minval: Value=KOUTP_ID2messageALTU_raw8_minval
      link override Signal_Override/_ovrdflg: Value=KOUTP_ID2messageALTU_raw8_ovrdflg
      link override Signal_Override/_ovrdval: Value=KOUTP_ID2messageALTU_raw8_ovrdval
  VTPM_ID3messageALTU_raw8_Inproc : FVT_lib/outp/OverrideAndLimit  SystemSampleTime=-1  VariantActivationTime=update diagram  Latency=0  AutoFrameSizeCalculation=off
      link override Signal_Limit/_maxval: Value=KOUTP_ID3messageALTU_raw8_maxval
      link override Signal_Limit/_minval: Value=KOUTP_ID3messageALTU_raw8_minval
      link override Signal_Override/_ovrdflg: Value=KOUTP_ID3messageALTU_raw8_ovrdflg
      link override Signal_Override/_ovrdval: Value=KOUTP_ID3messageALTU_raw8_ovrdval
  VTPM_ID4messageALTU_raw8_Inproc : FVT_lib/outp/OverrideAndLimit  SystemSampleTime=-1  VariantActivationTime=update diagram  Latency=0  AutoFrameSizeCalculation=off
      link override Signal_Limit/_maxval: Value=KOUTP_ID4messageALTU_raw8_maxval
      link override Signal_Limit/_minval: Value=KOUTP_ID4messageALTU_raw8_minval
      link override Signal_Override/_ovrdflg: Value=KOUTP_ID4messageALTU_raw8_ovrdflg
      link override Signal_Override/_ovrdval: Value=KOUTP_ID4messageALTU_raw8_ovrdval
  VTPM_IDin_raw32_Inproc : FVT_lib/outp/OverrideAndLimit  SystemSampleTime=-1  VariantActivationTime=update diagram  Latency=0  AutoFrameSizeCalculation=off
      link override Signal_Limit/_maxval: Value=KOUTP_IDin_raw32_maxval
      link override Signal_Limit/_minval: Value=KOUTP_IDin_raw32_minval
      link override Signal_Override/_ovrdflg: Value=KOUTP_IDin_raw32_ovrdflg
      link override Signal_Override/_ovrdval: Value=KOUTP_IDin_raw32_ovrdval
  VTPM_LFBatWarn_flg_Inproc : FVT_lib/outp/OverrideAndLimit  SystemSampleTime=-1  VariantActivationTime=update diagram  Latency=0  AutoFrameSizeCalculation=off
      link override Signal_Limit/_maxval: Value=KOUTP_LFBatWarn_flg_maxval
      link override Signal_Limit/_minval: Value=KOUTP_LFBatWarn_flg_minval
      link override Signal_Override/_ovrdflg: Value=KOUTP_LFBatWarn_flg_ovrdflg
      link override Signal_Override/_ovrdval: Value=KOUTP_LFBatWarn_flg_ovrdval
  VTPM_LFP20_raw8_Inproc : FVT_lib/outp/OverrideAndLimit  SystemSampleTime=-1  VariantActivationTime=update diagram  Latency=0  AutoFrameSizeCalculation=off
      link override Signal_Limit/_maxval: Value=KOUTP_LFP20_raw8_maxval
      link override Signal_Limit/_minval: Value=KOUTP_LFP20_raw8_minval
      link override Signal_Override/_ovrdflg: Value=KOUTP_LFP20_raw8_ovrdflg
      link override Signal_Override/_ovrdval: Value=KOUTP_LFP20_raw8_ovrdval
  VTPM_LFPindi_enum_Inproc : FVT_lib/outp/OverrideAndLimit  SystemSampleTime=-1  VariantActivationTime=update diagram  Latency=0  AutoFrameSizeCalculation=off
      link override Signal_Limit/_maxval: Value=KOUTP_LFPindi_enum_maxval
      link override Signal_Limit/_minval: Value=KOUTP_LFPindi_enum_minval
      link override Signal_Override/_ovrdflg: Value=KOUTP_LFPindi_enum_ovrdflg
      link override Signal_Override/_ovrdval: Value=KOUTP_LFPindi_enum_ovrdval
  VTPM_LFPressIndi_enum_Inproc : FVT_lib/outp/OverrideAndLimit  SystemSampleTime=-1  VariantActivationTime=update diagram  Latency=0  AutoFrameSizeCalculation=off
      link override Signal_Limit/_maxval: Value=KOUTP_LFPressIndi_enum_maxval
      link override Signal_Limit/_minval: Value=KOUTP_LFPressIndi_enum_minval
      link override Signal_Override/_ovrdflg: Value=KOUTP_LFPressIndi_enum_ovrdflg
      link override Signal_Override/_ovrdval: Value=KOUTP_LFPressIndi_enum_ovrdval
  VTPM_LFSensorFail_flg_Inproc : FVT_lib/outp/OverrideAndLimit  SystemSampleTime=-1  VariantActivationTime=update diagram  Latency=0  AutoFrameSizeCalculation=off
      link override Signal_Limit/_maxval: Value=KOUTP_LFSensorFail_flg_maxval
      link override Signal_Limit/_minval: Value=KOUTP_LFSensorFail_flg_minval
      link override Signal_Override/_ovrdflg: Value=KOUTP_LFSensorFail_flg_ovrdflg
      link override Signal_Override/_ovrdval: Value=KOUTP_LFSensorFail_flg_ovrdval
  VTPM_LFSensorMode_flg_Inproc : FVT_lib/outp/OverrideAndLimit  SystemSampleTime=-1  VariantActivationTime=update diagram  Latency=0  AutoFrameSizeCalculation=off
      link override Signal_Limit/_maxval: Value=KOUTP_LFSensorMode_flg_maxval
      link override Signal_Limit/_minval: Value=KOUTP_LFSensorMode_flg_minval
      link override Signal_Override/_ovrdflg: Value=KOUTP_LFSensorMode_flg_ovrdflg
      link override Signal_Override/_ovrdval: Value=KOUTP_LFSensorMode_flg_ovrdval
  VTPM_LFWheelDebug_flg_Inproc : FVT_lib/outp/OverrideAndLimit  SystemSampleTime=-1  VariantActivationTime=update diagram  Latency=0  AutoFrameSizeCalculation=off
      link override Signal_Limit/_maxval: Value=KOUTP_LFWheelDebug_flg_maxval
      link override Signal_Limit/_minval: Value=KOUTP_LFWheelDebug_flg_minval
      link override Signal_Override/_ovrdflg: Value=KOUTP_LFWheelDebug_flg_ovrdflg
      link override Signal_Override/_ovrdval: Value=KOUTP_LFWheelDebug_flg_ovrdval
  VTPM_LFWheelPSW_raw8_Inproc : FVT_lib/outp/OverrideAndLimit  SystemSampleTime=-1  VariantActivationTime=update diagram  Latency=0  AutoFrameSizeCalculation=off
      link override Signal_Limit/_maxval: Value=KOUTP_LFWheelPSW_raw8_maxval
      link override Signal_Limit/_minval: Value=KOUTP_LFWheelPSW_raw8_minval
      link override Signal_Override/_ovrdflg: Value=KOUTP_LFWheelPSW_raw8_ovrdflg
      link override Signal_Override/_ovrdval: Value=KOUTP_LFWheelPSW_raw8_ovrdval
  VTPM_LFWheelPress_raw8_Inproc : FVT_lib/outp/OverrideAndLimit  SystemSampleTime=-1  VariantActivationTime=update diagram  Latency=0  AutoFrameSizeCalculation=off
      link override Signal_Limit/_maxval: Value=KOUTP_LFWheelPress_raw8_maxval
      link override Signal_Limit/_minval: Value=KOUTP_LFWheelPress_raw8_minval
      link override Signal_Override/_ovrdflg: Value=KOUTP_LFWheelPress_raw8_ovrdflg
      link override Signal_Override/_ovrdval: Value=KOUTP_LFWheelPress_raw8_ovrdval
  VTPM_LFWheelTemp_C_Inproc : FVT_lib/outp/OverrideAndLimit  SystemSampleTime=-1  VariantActivationTime=update diagram  Latency=0  AutoFrameSizeCalculation=off
      link override Signal_Limit/_maxval: Value=KOUTP_LFWheelTemp_C_maxval
      link override Signal_Limit/_minval: Value=KOUTP_LFWheelTemp_C_minval
      link override Signal_Override/_ovrdflg: Value=KOUTP_LFWheelTemp_C_ovrdflg
      link override Signal_Override/_ovrdval: Value=KOUTP_LFWheelTemp_C_ovrdval
  VTPM_LFWheelTmpIndi_flg_Inproc : FVT_lib/outp/OverrideAndLimit  SystemSampleTime=-1  VariantActivationTime=update diagram  Latency=0  AutoFrameSizeCalculation=off
      link override Signal_Limit/_maxval: Value=KOUTP_LFWheelTmpIndi_flg_maxval
      link override Signal_Limit/_minval: Value=KOUTP_LFWheelTmpIndi_flg_minval
      link override Signal_Override/_ovrdflg: Value=KOUTP_LFWheelTmpIndi_flg_ovrdflg
      link override Signal_Override/_ovrdval: Value=KOUTP_LFWheelTmpIndi_flg_ovrdval
  VTPM_LProgress_enum_Inproc : FVT_lib/outp/OverrideAndLimit  SystemSampleTime=-1  VariantActivationTime=update diagram  Latency=0  AutoFrameSizeCalculation=off
      link override Signal_Limit/_maxval: Value=KOUTP_LProgress_enum_maxval
      link override Signal_Limit/_minval: Value=KOUTP_LProgress_enum_minval
      link override Signal_Override/_ovrdflg: Value=KOUTP_LProgress_enum_ovrdflg
      link override Signal_Override/_ovrdval: Value=KOUTP_LProgress_enum_ovrdval
  VTPM_LRBatWarn_flg_Inproc : FVT_lib/outp/OverrideAndLimit  SystemSampleTime=-1  VariantActivationTime=update diagram  Latency=0  AutoFrameSizeCalculation=off
      link override Signal_Limit/_maxval: Value=KOUTP_LRBatWarn_flg_maxval
      link override Signal_Limit/_minval: Value=KOUTP_LRBatWarn_flg_minval
      link override Signal_Override/_ovrdflg: Value=KOUTP_LRBatWarn_flg_ovrdflg
      link override Signal_Override/_ovrdval: Value=KOUTP_LRBatWarn_flg_ovrdval
  VTPM_LRP20_raw8_Inproc : FVT_lib/outp/OverrideAndLimit  SystemSampleTime=-1  VariantActivationTime=update diagram  Latency=0  AutoFrameSizeCalculation=off
      link override Signal_Limit/_maxval: Value=KOUTP_LRP20_raw8_maxval
      link override Signal_Limit/_minval: Value=KOUTP_LRP20_raw8_minval
      link override Signal_Override/_ovrdflg: Value=KOUTP_LRP20_raw8_ovrdflg
      link override Signal_Override/_ovrdval: Value=KOUTP_LRP20_raw8_ovrdval
  VTPM_LRPindi_enum_Inproc : FVT_lib/outp/OverrideAndLimit  SystemSampleTime=-1  VariantActivationTime=update diagram  Latency=0  AutoFrameSizeCalculation=off
      link override Signal_Limit/_maxval: Value=KOUTP_LRPindi_enum_maxval
      link override Signal_Limit/_minval: Value=KOUTP_LRPindi_enum_minval
      link override Signal_Override/_ovrdflg: Value=KOUTP_LRPindi_enum_ovrdflg
      link override Signal_Override/_ovrdval: Value=KOUTP_LRPindi_enum_ovrdval
  VTPM_LRPressIndi_enum_Inproc : FVT_lib/outp/OverrideAndLimit  SystemSampleTime=-1  VariantActivationTime=update diagram  Latency=0  AutoFrameSizeCalculation=off
      link override Signal_Limit/_maxval: Value=KOUTP_LRPressIndi_enum_maxval
      link override Signal_Limit/_minval: Value=KOUTP_LRPressIndi_enum_minval
      link override Signal_Override/_ovrdflg: Value=KOUTP_LRPressIndi_enum_ovrdflg
      link override Signal_Override/_ovrdval: Value=KOUTP_LRPressIndi_enum_ovrdval
  VTPM_LRSensorFail_flg_Inproc : FVT_lib/outp/OverrideAndLimit  SystemSampleTime=-1  VariantActivationTime=update diagram  Latency=0  AutoFrameSizeCalculation=off
      link override Signal_Limit/_maxval: Value=KOUTP_LRSensorFail_flg_maxval
      link override Signal_Limit/_minval: Value=KOUTP_LRSensorFail_flg_minval
      link override Signal_Override/_ovrdflg: Value=KOUTP_LRSensorFail_flg_ovrdflg
      link override Signal_Override/_ovrdval: Value=KOUTP_LRSensorFail_flg_ovrdval
  VTPM_LRSensorMode_flg_Inproc : FVT_lib/outp/OverrideAndLimit  SystemSampleTime=-1  VariantActivationTime=update diagram  Latency=0  AutoFrameSizeCalculation=off
      link override Signal_Limit/_maxval: Value=KOUTP_LRSensorMode_flg_maxval
      link override Signal_Limit/_minval: Value=KOUTP_LRSensorMode_flg_minval
      link override Signal_Override/_ovrdflg: Value=KOUTP_LRSensorMode_flg_ovrdflg
      link override Signal_Override/_ovrdval: Value=KOUTP_LRSensorMode_flg_ovrdval
  VTPM_LRWheelDebug_flg_Inproc : FVT_lib/outp/OverrideAndLimit  SystemSampleTime=-1  VariantActivationTime=update diagram  Latency=0  AutoFrameSizeCalculation=off
      link override Signal_Limit/_maxval: Value=KOUTP_LRWheelDebug_flg_maxval
      link override Signal_Limit/_minval: Value=KOUTP_LRWheelDebug_flg_minval
      link override Signal_Override/_ovrdflg: Value=KOUTP_LRWheelDebug_flg_ovrdflg
      link override Signal_Override/_ovrdval: Value=KOUTP_LRWheelDebug_flg_ovrdval
  VTPM_LRWheelPSW_raw8_Inproc : FVT_lib/outp/OverrideAndLimit  SystemSampleTime=-1  VariantActivationTime=update diagram  Latency=0  AutoFrameSizeCalculation=off
      link override Signal_Limit/_maxval: Value=KOUTP_LRWheelPSW_raw8_maxval
      link override Signal_Limit/_minval: Value=KOUTP_LRWheelPSW_raw8_minval
      link override Signal_Override/_ovrdflg: Value=KOUTP_LRWheelPSW_raw8_ovrdflg
      link override Signal_Override/_ovrdval: Value=KOUTP_LRWheelPSW_raw8_ovrdval
  VTPM_LRWheelPress_raw8_Inproc : FVT_lib/outp/OverrideAndLimit  SystemSampleTime=-1  VariantActivationTime=update diagram  Latency=0  AutoFrameSizeCalculation=off
      link override Signal_Limit/_maxval: Value=KOUTP_LRWheelPress_raw8_maxval
      link override Signal_Limit/_minval: Value=KOUTP_LRWheelPress_raw8_minval
      link override Signal_Override/_ovrdflg: Value=KOUTP_LRWheelPress_raw8_ovrdflg
      link override Signal_Override/_ovrdval: Value=KOUTP_LRWheelPress_raw8_ovrdval
  VTPM_LRWheelTemp_C_Inproc : FVT_lib/outp/OverrideAndLimit  SystemSampleTime=-1  VariantActivationTime=update diagram  Latency=0  AutoFrameSizeCalculation=off
      link override Signal_Limit/_maxval: Value=KOUTP_LRWheelTemp_C_maxval
      link override Signal_Limit/_minval: Value=KOUTP_LRWheelTemp_C_minval
      link override Signal_Override/_ovrdflg: Value=KOUTP_LRWheelTemp_C_ovrdflg
      link override Signal_Override/_ovrdval: Value=KOUTP_LRWheelTemp_C_ovrdval
  VTPM_LRWheelTmpIndi_flg_Inproc : FVT_lib/outp/OverrideAndLimit  SystemSampleTime=-1  VariantActivationTime=update diagram  Latency=0  AutoFrameSizeCalculation=off
      link override Signal_Limit/_maxval: Value=KOUTP_LRWheelTmpIndi_flg_maxval
      link override Signal_Limit/_minval: Value=KOUTP_LRWheelTmpIndi_flg_minval
      link override Signal_Override/_ovrdflg: Value=KOUTP_LRWheelTmpIndi_flg_ovrdflg
      link override Signal_Override/_ovrdval: Value=KOUTP_LRWheelTmpIndi_flg_ovrdval
  VTPM_ModelVersionChksum_raw_Inproc : FVT_lib/outp/OverrideAndLimit  SystemSampleTime=-1  VariantActivationTime=update diagram  Latency=0  AutoFrameSizeCalculation=off
      link override Signal_Limit/_maxval: Value=KOUTP_ModelVersionChksum_raw_maxval
      link override Signal_Limit/_minval: Value=KOUTP_ModelVersionChksum_raw_minval
      link override Signal_Override/_ovrdflg: Value=KOUTP_ModelVersionChksum_raw_ovrdflg
      link override Signal_Override/_ovrdval: Value=KOUTP_ModelVersionChksum_raw_ovrdval
  VTPM_ModelVersion_raw_Inproc : FVT_lib/outp/OverrideAndLimit  SystemSampleTime=-1  VariantActivationTime=update diagram  Latency=0  AutoFrameSizeCalculation=off
      link override Signal_Limit/_maxval: Value=KOUTP_ModelVersion_raw_maxval
      link override Signal_Limit/_minval: Value=KOUTP_ModelVersion_raw_minval
      link override Signal_Override/_ovrdflg: Value=KOUTP_ModelVersion_raw_ovrdflg
      link override Signal_Override/_ovrdval: Value=KOUTP_ModelVersion_raw_ovrdval
  VTPM_Prepresstempvalid_enum_Inproc : FVT_lib/outp/OverrideAndLimit  SystemSampleTime=-1  VariantActivationTime=update diagram  Latency=0  AutoFrameSizeCalculation=off
      link override Signal_Limit/_maxval: Value=KOUTP_Prepresstempvalid_enum_maxval
      link override Signal_Limit/_minval: Value=KOUTP_Prepresstempvalid_enum_minval
      link override Signal_Override/_ovrdflg: Value=KOUTP_Prepresstempvalid_enum_ovrdflg
      link override Signal_Override/_ovrdval: Value=KOUTP_Prepresstempvalid_enum_ovrdval
  VTPM_RFBatWarn_flg_Inproc : FVT_lib/outp/OverrideAndLimit  SystemSampleTime=-1  VariantActivationTime=update diagram  Latency=0  AutoFrameSizeCalculation=off
      link override Signal_Limit/_maxval: Value=KOUTP_RFBatWarn_flg_maxval
      link override Signal_Limit/_minval: Value=KOUTP_RFBatWarn_flg_minval
      link override Signal_Override/_ovrdflg: Value=KOUTP_RFBatWarn_flg_ovrdflg
      link override Signal_Override/_ovrdval: Value=KOUTP_RFBatWarn_flg_ovrdval
  VTPM_RFP20_raw8_Inproc : FVT_lib/outp/OverrideAndLimit  SystemSampleTime=-1  VariantActivationTime=update diagram  Latency=0  AutoFrameSizeCalculation=off
      link override Signal_Limit/_maxval: Value=KOUTP_RFP20_raw8_maxval
      link override Signal_Limit/_minval: Value=KOUTP_RFP20_raw8_minval
      link override Signal_Override/_ovrdflg: Value=KOUTP_RFP20_raw8_ovrdflg
      link override Signal_Override/_ovrdval: Value=KOUTP_RFP20_raw8_ovrdval
  VTPM_RFPind_enum_Inproc : FVT_lib/outp/OverrideAndLimit  SystemSampleTime=-1  VariantActivationTime=update diagram  Latency=0  AutoFrameSizeCalculation=off
      link override Signal_Limit/_maxval: Value=KOUTP_RFPind_enum_maxval
      link override Signal_Limit/_minval: Value=KOUTP_RFPind_enum_minval
      link override Signal_Override/_ovrdflg: Value=KOUTP_RFPind_enum_ovrdflg
      link override Signal_Override/_ovrdval: Value=KOUTP_RFPind_enum_ovrdval
  VTPM_RFPressIndi_enum_Inproc : FVT_lib/outp/OverrideAndLimit  SystemSampleTime=-1  VariantActivationTime=update diagram  Latency=0  AutoFrameSizeCalculation=off
      link override Signal_Limit/_maxval: Value=KOUTP_RFPressIndi_enum_maxval
      link override Signal_Limit/_minval: Value=KOUTP_RFPressIndi_enum_minval
      link override Signal_Override/_ovrdflg: Value=KOUTP_RFPressIndi_enum_ovrdflg
      link override Signal_Override/_ovrdval: Value=KOUTP_RFPressIndi_enum_ovrdval
  VTPM_RFSensorFail_flg_Inproc : FVT_lib/outp/OverrideAndLimit  SystemSampleTime=-1  VariantActivationTime=update diagram  Latency=0  AutoFrameSizeCalculation=off
      link override Signal_Limit/_maxval: Value=KOUTP_RFSensorFail_flg_maxval
      link override Signal_Limit/_minval: Value=KOUTP_RFSensorFail_flg_minval
      link override Signal_Override/_ovrdflg: Value=KOUTP_RFSensorFail_flg_ovrdflg
      link override Signal_Override/_ovrdval: Value=KOUTP_RFSensorFail_flg_ovrdval
  VTPM_RFSensorMode_flg_Inproc : FVT_lib/outp/OverrideAndLimit  SystemSampleTime=-1  VariantActivationTime=update diagram  Latency=0  AutoFrameSizeCalculation=off
      link override Signal_Limit/_maxval: Value=KOUTP_RFSensorMode_flg_maxval
      link override Signal_Limit/_minval: Value=KOUTP_RFSensorMode_flg_minval
      link override Signal_Override/_ovrdflg: Value=KOUTP_RFSensorMode_flg_ovrdflg
      link override Signal_Override/_ovrdval: Value=KOUTP_RFSensorMode_flg_ovrdval
  VTPM_RFWheelDebug_flg_Inproc : FVT_lib/outp/OverrideAndLimit  SystemSampleTime=-1  VariantActivationTime=update diagram  Latency=0  AutoFrameSizeCalculation=off
      link override Signal_Limit/_maxval: Value=KOUTP_RFWheelDebug_flg_maxval
      link override Signal_Limit/_minval: Value=KOUTP_RFWheelDebug_flg_minval
      link override Signal_Override/_ovrdflg: Value=KOUTP_RFWheelDebug_flg_ovrdflg
      link override Signal_Override/_ovrdval: Value=KOUTP_RFWheelDebug_flg_ovrdval
  VTPM_RFWheelPSW_raw8_Inproc : FVT_lib/outp/OverrideAndLimit  SystemSampleTime=-1  VariantActivationTime=update diagram  Latency=0  AutoFrameSizeCalculation=off
      link override Signal_Limit/_maxval: Value=KOUTP_RFWheelPSW_raw8_maxval
      link override Signal_Limit/_minval: Value=KOUTP_RFWheelPSW_raw8_minval
      link override Signal_Override/_ovrdflg: Value=KOUTP_RFWheelPSW_raw8_ovrdflg
      link override Signal_Override/_ovrdval: Value=KOUTP_RFWheelPSW_raw8_ovrdval
  VTPM_RFWheelPress_raw8_Inproc : FVT_lib/outp/OverrideAndLimit  SystemSampleTime=-1  VariantActivationTime=update diagram  Latency=0  AutoFrameSizeCalculation=off
      link override Signal_Limit/_maxval: Value=KOUTP_RFWheelPress_raw8_maxval
      link override Signal_Limit/_minval: Value=KOUTP_RFWheelPress_raw8_minval
      link override Signal_Override/_ovrdflg: Value=KOUTP_RFWheelPress_raw8_ovrdflg
      link override Signal_Override/_ovrdval: Value=KOUTP_RFWheelPress_raw8_ovrdval
  VTPM_RFWheelTemp_C_Inproc : FVT_lib/outp/OverrideAndLimit  SystemSampleTime=-1  VariantActivationTime=update diagram  Latency=0  AutoFrameSizeCalculation=off
      link override Signal_Limit/_maxval: Value=KOUTP_RFWheelTemp_C_maxval
      link override Signal_Limit/_minval: Value=KOUTP_RFWheelTemp_C_minval
      link override Signal_Override/_ovrdflg: Value=KOUTP_RFWheelTemp_C_ovrdflg
      link override Signal_Override/_ovrdval: Value=KOUTP_RFWheelTemp_C_ovrdval
  VTPM_RFWheelTmpIndi_flg_Inproc : FVT_lib/outp/OverrideAndLimit  SystemSampleTime=-1  VariantActivationTime=update diagram  Latency=0  AutoFrameSizeCalculation=off
      link override Signal_Limit/_maxval: Value=KOUTP_RFWheelTmpIndi_flg_maxval
      link override Signal_Limit/_minval: Value=KOUTP_RFWheelTmpIndi_flg_minval
      link override Signal_Override/_ovrdflg: Value=KOUTP_RFWheelTmpIndi_flg_ovrdflg
      link override Signal_Override/_ovrdval: Value=KOUTP_RFWheelTmpIndi_flg_ovrdval
  VTPM_RRBatWarn_flg_Inproc : FVT_lib/outp/OverrideAndLimit  SystemSampleTime=-1  VariantActivationTime=update diagram  Latency=0  AutoFrameSizeCalculation=off
      link override Signal_Limit/_maxval: Value=KOUTP_RRBatWarn_flg_maxval
      link override Signal_Limit/_minval: Value=KOUTP_RRBatWarn_flg_minval
      link override Signal_Override/_ovrdflg: Value=KOUTP_RRBatWarn_flg_ovrdflg
      link override Signal_Override/_ovrdval: Value=KOUTP_RRBatWarn_flg_ovrdval
  VTPM_RRP20_raw8_Inproc : FVT_lib/outp/OverrideAndLimit  SystemSampleTime=-1  VariantActivationTime=update diagram  Latency=0  AutoFrameSizeCalculation=off
      link override Signal_Limit/_maxval: Value=KOUTP_RRP20_raw8_maxval
      link override Signal_Limit/_minval: Value=KOUTP_RRP20_raw8_minval
      link override Signal_Override/_ovrdflg: Value=KOUTP_RRP20_raw8_ovrdflg
      link override Signal_Override/_ovrdval: Value=KOUTP_RRP20_raw8_ovrdval
  VTPM_RRPindi_enum_Inproc : FVT_lib/outp/OverrideAndLimit  SystemSampleTime=-1  VariantActivationTime=update diagram  Latency=0  AutoFrameSizeCalculation=off
      link override Signal_Limit/_maxval: Value=KOUTP_RRPindi_enum_maxval
      link override Signal_Limit/_minval: Value=KOUTP_RRPindi_enum_minval
      link override Signal_Override/_ovrdflg: Value=KOUTP_RRPindi_enum_ovrdflg
      link override Signal_Override/_ovrdval: Value=KOUTP_RRPindi_enum_ovrdval
  VTPM_RRPressIndi_enum_Inproc : FVT_lib/outp/OverrideAndLimit  SystemSampleTime=-1  VariantActivationTime=update diagram  Latency=0  AutoFrameSizeCalculation=off
      link override Signal_Limit/_maxval: Value=KOUTP_RRPressIndi_enum_maxval
      link override Signal_Limit/_minval: Value=KOUTP_RRPressIndi_enum_minval
      link override Signal_Override/_ovrdflg: Value=KOUTP_RRPressIndi_enum_ovrdflg
      link override Signal_Override/_ovrdval: Value=KOUTP_RRPressIndi_enum_ovrdval
  VTPM_RRSensorFail_flg_Inproc : FVT_lib/outp/OverrideAndLimit  SystemSampleTime=-1  VariantActivationTime=update diagram  Latency=0  AutoFrameSizeCalculation=off
      link override Signal_Limit/_maxval: Value=KOUTP_RRSensorFail_flg_maxval
      link override Signal_Limit/_minval: Value=KOUTP_RRSensorFail_flg_minval
      link override Signal_Override/_ovrdflg: Value=KOUTP_RRSensorFail_flg_ovrdflg
      link override Signal_Override/_ovrdval: Value=KOUTP_RRSensorFail_flg_ovrdval
  VTPM_RRSensorMode_flg_Inproc : FVT_lib/outp/OverrideAndLimit  SystemSampleTime=-1  VariantActivationTime=update diagram  Latency=0  AutoFrameSizeCalculation=off
      link override Signal_Limit/_maxval: Value=KOUTP_RRSensorMode_flg_maxval
      link override Signal_Limit/_minval: Value=KOUTP_RRSensorMode_flg_minval
      link override Signal_Override/_ovrdflg: Value=KOUTP_RRSensorMode_flg_ovrdflg
      link override Signal_Override/_ovrdval: Value=KOUTP_RRSensorMode_flg_ovrdval
  VTPM_RRWheelDebug_flg_Inproc : FVT_lib/outp/OverrideAndLimit  SystemSampleTime=-1  VariantActivationTime=update diagram  Latency=0  AutoFrameSizeCalculation=off
      link override Signal_Limit/_maxval: Value=KOUTP_RRWheelDebug_flg_maxval
      link override Signal_Limit/_minval: Value=KOUTP_RRWheelDebug_flg_minval
      link override Signal_Override/_ovrdflg: Value=KOUTP_RRWheelDebug_flg_ovrdflg
      link override Signal_Override/_ovrdval: Value=KOUTP_RRWheelDebug_flg_ovrdval
  VTPM_RRWheelPSW_raw8_Inproc : FVT_lib/outp/OverrideAndLimit  SystemSampleTime=-1  VariantActivationTime=update diagram  Latency=0  AutoFrameSizeCalculation=off
      link override Signal_Limit/_maxval: Value=KOUTP_RRWheelPSW_raw8_maxval
      link override Signal_Limit/_minval: Value=KOUTP_RRWheelPSW_raw8_minval
      link override Signal_Override/_ovrdflg: Value=KOUTP_RRWheelPSW_raw8_ovrdflg
      link override Signal_Override/_ovrdval: Value=KOUTP_RRWheelPSW_raw8_ovrdval
  VTPM_RRWheelPress_raw8_Inproc : FVT_lib/outp/OverrideAndLimit  SystemSampleTime=-1  VariantActivationTime=update diagram  Latency=0  AutoFrameSizeCalculation=off
      link override Signal_Limit/_maxval: Value=KOUTP_RRWheelPress_raw8_maxval
      link override Signal_Limit/_minval: Value=KOUTP_RRWheelPress_raw8_minval
      link override Signal_Override/_ovrdflg: Value=KOUTP_RRWheelPress_raw8_ovrdflg
      link override Signal_Override/_ovrdval: Value=KOUTP_RRWheelPress_raw8_ovrdval
  VTPM_RRWheelTemp_C_Inproc : FVT_lib/outp/OverrideAndLimit  SystemSampleTime=-1  VariantActivationTime=update diagram  Latency=0  AutoFrameSizeCalculation=off
      link override Signal_Limit/_maxval: Value=KOUTP_RRWheelTemp_C_maxval
      link override Signal_Limit/_minval: Value=KOUTP_RRWheelTemp_C_minval
      link override Signal_Override/_ovrdflg: Value=KOUTP_RRWheelTemp_C_ovrdflg
      link override Signal_Override/_ovrdval: Value=KOUTP_RRWheelTemp_C_ovrdval
  VTPM_RRWheelTmpIndi_flg_Inproc : FVT_lib/outp/OverrideAndLimit  SystemSampleTime=-1  VariantActivationTime=update diagram  Latency=0  AutoFrameSizeCalculation=off
      link override Signal_Limit/_maxval: Value=KOUTP_RRWheelTmpIndi_flg_maxval
      link override Signal_Limit/_minval: Value=KOUTP_RRWheelTmpIndi_flg_minval
      link override Signal_Override/_ovrdflg: Value=KOUTP_RRWheelTmpIndi_flg_ovrdflg
      link override Signal_Override/_ovrdval: Value=KOUTP_RRWheelTmpIndi_flg_ovrdval
  VTPM_S1ID_raw32_Inproc : FVT_lib/outp/OverrideAndLimit  SystemSampleTime=-1  VariantActivationTime=update diagram  Latency=0  AutoFrameSizeCalculation=off
      link override Signal_Limit/_maxval: Value=KOUTP_S1ID_raw32_maxval
      link override Signal_Limit/_minval: Value=KOUTP_S1ID_raw32_minval
      link override Signal_Override/_ovrdflg: Value=KOUTP_S1ID_raw32_ovrdflg
      link override Signal_Override/_ovrdval: Value=KOUTP_S1ID_raw32_ovrdval
  VTPM_S1L_enum_Inproc : FVT_lib/outp/OverrideAndLimit  SystemSampleTime=-1  VariantActivationTime=update diagram  Latency=0  AutoFrameSizeCalculation=off
      link override Signal_Limit/_maxval: Value=KOUTP_S1L_enum_maxval
      link override Signal_Limit/_minval: Value=KOUTP_S1L_enum_minval
      link override Signal_Override/_ovrdflg: Value=KOUTP_S1L_enum_ovrdflg
      link override Signal_Override/_ovrdval: Value=KOUTP_S1L_enum_ovrdval
  VTPM_S1WheelDebugALTU_pct_Inproc : FVT_lib/outp/OverrideAndLimit  SystemSampleTime=-1  VariantActivationTime=update diagram  Latency=0  AutoFrameSizeCalculation=off
      link override Signal_Limit/_maxval: Value=KOUTP_S1WheelDebugALTU_pct_maxval
      link override Signal_Limit/_minval: Value=KOUTP_S1WheelDebugALTU_pct_minval
      link override Signal_Override/_ovrdflg: Value=KOUTP_S1WheelDebugALTU_pct_ovrdflg
      link override Signal_Override/_ovrdval: Value=KOUTP_S1WheelDebugALTU_pct_ovrdval
  VTPM_S2ID_raw32_Inproc : FVT_lib/outp/OverrideAndLimit  SystemSampleTime=-1  VariantActivationTime=update diagram  Latency=0  AutoFrameSizeCalculation=off
      link override Signal_Limit/_maxval: Value=KOUTP_S2ID_raw32_maxval
      link override Signal_Limit/_minval: Value=KOUTP_S2ID_raw32_minval
      link override Signal_Override/_ovrdflg: Value=KOUTP_S2ID_raw32_ovrdflg
      link override Signal_Override/_ovrdval: Value=KOUTP_S2ID_raw32_ovrdval
  VTPM_S2L_enum_Inproc : FVT_lib/outp/OverrideAndLimit  SystemSampleTime=-1  VariantActivationTime=update diagram  Latency=0  AutoFrameSizeCalculation=off
      link override Signal_Limit/_maxval: Value=KOUTP_S2L_enum_maxval
      link override Signal_Limit/_minval: Value=KOUTP_S2L_enum_minval
      link override Signal_Override/_ovrdflg: Value=KOUTP_S2L_enum_ovrdflg
      link override Signal_Override/_ovrdval: Value=KOUTP_S2L_enum_ovrdval
  VTPM_S2WheelDebugALTU_pct_Inproc : FVT_lib/outp/OverrideAndLimit  SystemSampleTime=-1  VariantActivationTime=update diagram  Latency=0  AutoFrameSizeCalculation=off
      link override Signal_Limit/_maxval: Value=KOUTP_S2WheelDebugALTU_pct_maxval
      link override Signal_Limit/_minval: Value=KOUTP_S2WheelDebugALTU_pct_minval
      link override Signal_Override/_ovrdflg: Value=KOUTP_S2WheelDebugALTU_pct_ovrdflg
      link override Signal_Override/_ovrdval: Value=KOUTP_S2WheelDebugALTU_pct_ovrdval
  VTPM_S3ID_raw32_Inproc : FVT_lib/outp/OverrideAndLimit  SystemSampleTime=-1  VariantActivationTime=update diagram  Latency=0  AutoFrameSizeCalculation=off
      link override Signal_Limit/_maxval: Value=KOUTP_S3ID_raw32_maxval
      link override Signal_Limit/_minval: Value=KOUTP_S3ID_raw32_minval
      link override Signal_Override/_ovrdflg: Value=KOUTP_S3ID_raw32_ovrdflg
      link override Signal_Override/_ovrdval: Value=KOUTP_S3ID_raw32_ovrdval
  VTPM_S3L_enum_Inproc : FVT_lib/outp/OverrideAndLimit  SystemSampleTime=-1  VariantActivationTime=update diagram  Latency=0  AutoFrameSizeCalculation=off
      link override Signal_Limit/_maxval: Value=KOUTP_S3L_enum_maxval
      link override Signal_Limit/_minval: Value=KOUTP_S3L_enum_minval
      link override Signal_Override/_ovrdflg: Value=KOUTP_S3L_enum_ovrdflg
      link override Signal_Override/_ovrdval: Value=KOUTP_S3L_enum_ovrdval
  VTPM_S3WheelDebugALTU_pct_Inproc : FVT_lib/outp/OverrideAndLimit  SystemSampleTime=-1  VariantActivationTime=update diagram  Latency=0  AutoFrameSizeCalculation=off
      link override Signal_Limit/_maxval: Value=KOUTP_S3WheelDebugALTU_pct_maxval
      link override Signal_Limit/_minval: Value=KOUTP_S3WheelDebugALTU_pct_minval
      link override Signal_Override/_ovrdflg: Value=KOUTP_S3WheelDebugALTU_pct_ovrdflg
      link override Signal_Override/_ovrdval: Value=KOUTP_S3WheelDebugALTU_pct_ovrdval
  VTPM_S4ID_raw32_Inproc : FVT_lib/outp/OverrideAndLimit  SystemSampleTime=-1  VariantActivationTime=update diagram  Latency=0  AutoFrameSizeCalculation=off
      link override Signal_Limit/_maxval: Value=KOUTP_S4ID_raw32_maxval
      link override Signal_Limit/_minval: Value=KOUTP_S4ID_raw32_minval
      link override Signal_Override/_ovrdflg: Value=KOUTP_S4ID_raw32_ovrdflg
      link override Signal_Override/_ovrdval: Value=KOUTP_S4ID_raw32_ovrdval
  VTPM_S4L_enum_Inproc : FVT_lib/outp/OverrideAndLimit  SystemSampleTime=-1  VariantActivationTime=update diagram  Latency=0  AutoFrameSizeCalculation=off
      link override Signal_Limit/_maxval: Value=KOUTP_S4L_enum_maxval
      link override Signal_Limit/_minval: Value=KOUTP_S4L_enum_minval
      link override Signal_Override/_ovrdflg: Value=KOUTP_S4L_enum_ovrdflg
      link override Signal_Override/_ovrdval: Value=KOUTP_S4L_enum_ovrdval
  VTPM_S4WheelDebugALTU_pct_Inproc : FVT_lib/outp/OverrideAndLimit  SystemSampleTime=-1  VariantActivationTime=update diagram  Latency=0  AutoFrameSizeCalculation=off
      link override Signal_Limit/_maxval: Value=KOUTP_S4WheelDebugALTU_pct_maxval
      link override Signal_Limit/_minval: Value=KOUTP_S4WheelDebugALTU_pct_minval
      link override Signal_Override/_ovrdflg: Value=KOUTP_S4WheelDebugALTU_pct_ovrdflg
      link override Signal_Override/_ovrdval: Value=KOUTP_S4WheelDebugALTU_pct_ovrdval
  VTPM_SetIDLoc_flg_Inproc : FVT_lib/outp/OverrideAndLimit  SystemSampleTime=-1  VariantActivationTime=update diagram  Latency=0  AutoFrameSizeCalculation=off
      link override Signal_Limit/_maxval: Value=KOUTP_SetIDLoc_flg_maxval
      link override Signal_Limit/_minval: Value=KOUTP_SetIDLoc_flg_minval
      link override Signal_Override/_ovrdflg: Value=KOUTP_SetIDLoc_flg_ovrdflg
      link override Signal_Override/_ovrdval: Value=KOUTP_SetIDLoc_flg_ovrdval
  VTPM_TPMSCaliButtAllow_flg_Inproc : FVT_lib/outp/OverrideAndLimit  SystemSampleTime=-1  VariantActivationTime=update diagram  Latency=0  AutoFrameSizeCalculation=off
      link override Signal_Limit/_maxval: Value=KOUTP_TPMSCaliButtAllow_flg_maxval
      link override Signal_Limit/_minval: Value=KOUTP_TPMSCaliButtAllow_flg_minval
      link override Signal_Override/_ovrdflg: Value=KOUTP_TPMSCaliButtAllow_flg_ovrdflg
      link override Signal_Override/_ovrdval: Value=KOUTP_TPMSCaliButtAllow_flg_ovrdval
  VTPM_TPMSResButtAllow_flg_Inproc : FVT_lib/outp/OverrideAndLimit  SystemSampleTime=-1  VariantActivationTime=update diagram  Latency=0  AutoFrameSizeCalculation=off
      link override Signal_Limit/_maxval: Value=KOUTP_TPMSResButtAllow_flg_maxval
      link override Signal_Limit/_minval: Value=KOUTP_TPMSResButtAllow_flg_minval
      link override Signal_Override/_ovrdflg: Value=KOUTP_TPMSResButtAllow_flg_ovrdflg
      link override Signal_Override/_ovrdval: Value=KOUTP_TPMSResButtAllow_flg_ovrdval
  VTPM_TPMSResButt_flg_Inproc : FVT_lib/outp/OverrideAndLimit  SystemSampleTime=-1  VariantActivationTime=update diagram  Latency=0  AutoFrameSizeCalculation=off
      link override Signal_Limit/_maxval: Value=KOUTP_TPMSResButt_flg_maxval
      link override Signal_Limit/_minval: Value=KOUTP_TPMSResButt_flg_minval
      link override Signal_Override/_ovrdflg: Value=KOUTP_TPMSResButt_flg_ovrdflg
      link override Signal_Override/_ovrdval: Value=KOUTP_TPMSResButt_flg_ovrdval
  VTPM_TPMSSensorIDRegStart_flg_Inproc : FVT_lib/outp/OverrideAndLimit  SystemSampleTime=-1  VariantActivationTime=update diagram  Latency=0  AutoFrameSizeCalculation=off
      link override Signal_Limit/_maxval: Value=KOUTP_TPMSSensorIDRegStart_flg_maxval
      link override Signal_Limit/_minval: Value=KOUTP_TPMSSensorIDRegStart_flg_minval
      link override Signal_Override/_ovrdflg: Value=KOUTP_TPMSSensorIDRegStart_flg_ovrdflg
      link override Signal_Override/_ovrdval: Value=KOUTP_TPMSSensorIDRegStart_flg_ovrdval
  VTPM_TPMSStorge_flg_Inproc : FVT_lib/outp/OverrideAndLimit  SystemSampleTime=-1  VariantActivationTime=update diagram  Latency=0  AutoFrameSizeCalculation=off
      link override Signal_Limit/_maxval: Value=KOUTP_TPMSStorge_flg_maxval
      link override Signal_Limit/_minval: Value=KOUTP_TPMSStorge_flg_minval
      link override Signal_Override/_ovrdflg: Value=KOUTP_TPMSStorge_flg_ovrdflg
      link override Signal_Override/_ovrdval: Value=KOUTP_TPMSStorge_flg_ovrdval
  VTPM_TPMSTLCmd_flg_Inproc : FVT_lib/outp/OverrideAndLimit  SystemSampleTime=-1  VariantActivationTime=update diagram  Latency=0  AutoFrameSizeCalculation=off
      link override Signal_Limit/_maxval: Value=KOUTP_TPMSTLCmd_flg_maxval
      link override Signal_Limit/_minval: Value=KOUTP_TPMSTLCmd_flg_minval
      link override Signal_Override/_ovrdflg: Value=KOUTP_TPMSTLCmd_flg_ovrdflg
      link override Signal_Override/_ovrdval: Value=KOUTP_TPMSTLCmd_flg_ovrdval
  VTPM_TPMSWarnIndi_enum_Inproc : FVT_lib/outp/OverrideAndLimit  SystemSampleTime=-1  VariantActivationTime=update diagram  Latency=0  AutoFrameSizeCalculation=off
      link override Signal_Limit/_maxval: Value=KOUTP_TPMSWarnIndi_enum_maxval
      link override Signal_Limit/_minval: Value=KOUTP_TPMSWarnIndi_enum_minval
      link override Signal_Override/_ovrdflg: Value=KOUTP_TPMSWarnIndi_enum_ovrdflg
      link override Signal_Override/_ovrdval: Value=KOUTP_TPMSWarnIndi_enum_ovrdval
  VTPM_WriteChkLFID_raw_Inproc : FVT_lib/outp/OverrideAndLimit  SystemSampleTime=-1  VariantActivationTime=update diagram  Latency=0  AutoFrameSizeCalculation=off
      link override Signal_Limit/_maxval: Value=KOUTP_WriteChkLFID_raw_maxval
      link override Signal_Limit/_minval: Value=KOUTP_WriteChkLFID_raw_minval
      link override Signal_Override/_ovrdflg: Value=KOUTP_WriteChkLFID_raw_ovrdflg
      link override Signal_Override/_ovrdval: Value=KOUTP_WriteChkLFID_raw_ovrdval
  VTPM_WriteChkLRID_raw_Inproc : FVT_lib/outp/OverrideAndLimit  SystemSampleTime=-1  VariantActivationTime=update diagram  Latency=0  AutoFrameSizeCalculation=off
      link override Signal_Limit/_maxval: Value=KOUTP_WriteChkLRID_raw_maxval
      link override Signal_Limit/_minval: Value=KOUTP_WriteChkLRID_raw_minval
      link override Signal_Override/_ovrdflg: Value=KOUTP_WriteChkLRID_raw_ovrdflg
      link override Signal_Override/_ovrdval: Value=KOUTP_WriteChkLRID_raw_ovrdval
  VTPM_WriteChkRFID_raw_Inproc : FVT_lib/outp/OverrideAndLimit  SystemSampleTime=-1  VariantActivationTime=update diagram  Latency=0  AutoFrameSizeCalculation=off
      link override Signal_Limit/_maxval: Value=KOUTP_WriteChkRFID_raw_maxval
      link override Signal_Limit/_minval: Value=KOUTP_WriteChkRFID_raw_minval
      link override Signal_Override/_ovrdflg: Value=KOUTP_WriteChkRFID_raw_ovrdflg
      link override Signal_Override/_ovrdval: Value=KOUTP_WriteChkRFID_raw_ovrdval
  VTPM_WriteChkRRID_raw_Inproc : FVT_lib/outp/OverrideAndLimit  SystemSampleTime=-1  VariantActivationTime=update diagram  Latency=0  AutoFrameSizeCalculation=off
      link override Signal_Limit/_maxval: Value=KOUTP_WriteChkRRID_raw_maxval
      link override Signal_Limit/_minval: Value=KOUTP_WriteChkRRID_raw_minval
      link override Signal_Override/_ovrdflg: Value=KOUTP_WriteChkRRID_raw_ovrdflg
      link override Signal_Override/_ovrdval: Value=KOUTP_WriteChkRRID_raw_ovrdval
  VTPM_WriteChkfinLFID_raw_Inproc : FVT_lib/outp/OverrideAndLimit  SystemSampleTime=-1  VariantActivationTime=update diagram  Latency=0  AutoFrameSizeCalculation=off
      link override Signal_Limit/_maxval: Value=KOUTP_WriteChkfinLFID_raw_maxval
      link override Signal_Limit/_minval: Value=KOUTP_WriteChkfinLFID_raw_minval
      link override Signal_Override/_ovrdflg: Value=KOUTP_WriteChkfinLFID_raw_ovrdflg
      link override Signal_Override/_ovrdval: Value=KOUTP_WriteChkfinLFID_raw_ovrdval
  VTPM_WriteChkfinLRID_raw_Inproc : FVT_lib/outp/OverrideAndLimit  SystemSampleTime=-1  VariantActivationTime=update diagram  Latency=0  AutoFrameSizeCalculation=off
      link override Signal_Limit/_maxval: Value=KOUTP_WriteChkfinLRID_raw_maxval
      link override Signal_Limit/_minval: Value=KOUTP_WriteChkfinLRID_raw_minval
      link override Signal_Override/_ovrdflg: Value=KOUTP_WriteChkfinLRID_raw_ovrdflg
      link override Signal_Override/_ovrdval: Value=KOUTP_WriteChkfinLRID_raw_ovrdval
  VTPM_WriteChkfinRFID_raw_Inproc : FVT_lib/outp/OverrideAndLimit  SystemSampleTime=-1  VariantActivationTime=update diagram  Latency=0  AutoFrameSizeCalculation=off
      link override Signal_Limit/_maxval: Value=KOUTP_WriteChkfinRFID_raw_maxval
      link override Signal_Limit/_minval: Value=KOUTP_WriteChkfinRFID_raw_minval
      link override Signal_Override/_ovrdflg: Value=KOUTP_WriteChkfinRFID_raw_ovrdflg
      link override Signal_Override/_ovrdval: Value=KOUTP_WriteChkfinRFID_raw_ovrdval
  VTPM_WriteChkfinRRID_raw_Inproc : FVT_lib/outp/OverrideAndLimit  SystemSampleTime=-1  VariantActivationTime=update diagram  Latency=0  AutoFrameSizeCalculation=off
      link override Signal_Limit/_maxval: Value=KOUTP_WriteChkfinRRID_raw_maxval
      link override Signal_Limit/_minval: Value=KOUTP_WriteChkfinRRID_raw_minval
      link override Signal_Override/_ovrdflg: Value=KOUTP_WriteChkfinRRID_raw_ovrdflg
      link override Signal_Override/_ovrdval: Value=KOUTP_WriteChkfinRRID_raw_ovrdval
  VTPM_WritingCnt_enum_Inproc : FVT_lib/outp/OverrideAndLimit  SystemSampleTime=-1  VariantActivationTime=update diagram  Latency=0  AutoFrameSizeCalculation=off
      link override Signal_Limit/_maxval: Value=KOUTP_WritingCnt_enum_maxval
      link override Signal_Limit/_minval: Value=KOUTP_WritingCnt_enum_minval
      link override Signal_Override/_ovrdflg: Value=KOUTP_WritingCnt_enum_ovrdflg
      link override Signal_Override/_ovrdval: Value=KOUTP_WritingCnt_enum_ovrdval
  VTPM_unlearnSfailvalid_enum_Inproc : FVT_lib/outp/OverrideAndLimit  SystemSampleTime=-1  VariantActivationTime=update diagram  Latency=0  AutoFrameSizeCalculation=off
      link override Signal_Limit/_maxval: Value=KOUTP_unlearnSfailvalid_enum_maxval
      link override Signal_Limit/_minval: Value=KOUTP_unlearnSfailvalid_enum_minval
      link override Signal_Override/_ovrdflg: Value=KOUTP_unlearnSfailvalid_enum_ovrdflg
      link override Signal_Override/_ovrdval: Value=KOUTP_unlearnSfailvalid_enum_ovrdval
  VTPM_unlearnSfali_flg_Inproc : FVT_lib/outp/OverrideAndLimit  SystemSampleTime=-1  VariantActivationTime=update diagram  Latency=0  AutoFrameSizeCalculation=off
      link override Signal_Limit/_maxval: Value=KOUTP_unlearnSfali_flg_maxval
      link override Signal_Limit/_minval: Value=KOUTP_unlearnSfali_flg_minval
      link override Signal_Override/_ovrdflg: Value=KOUTP_unlearnSfali_flg_ovrdflg
      link override Signal_Override/_ovrdval: Value=KOUTP_unlearnSfali_flg_ovrdval
  VTQD_ActDriveMode_enum_Inproc : FVT_lib/outp/OverrideAndLimit  SystemSampleTime=-1  VariantActivationTime=update diagram  Latency=0  AutoFrameSizeCalculation=off
      link override Signal_Limit/_maxval: Value=KOUTP_ActDriveMode_enum_maxval
      link override Signal_Limit/_minval: Value=KOUTP_ActDriveMode_enum_minval
      link override Signal_Override/_ovrdflg: Value=KOUTP_ActDriveMode_enum_ovrdflg
      link override Signal_Override/_ovrdval: Value=KOUTP_ActDriveMode_enum_ovrdval
  VTQD_ActTUpAIND_enum_Inproc : FVT_lib/outp/OverrideAndLimit  SystemSampleTime=-1  VariantActivationTime=update diagram  Latency=0  AutoFrameSizeCalculation=off
      link override Signal_Limit/_maxval: Value=KOUTP_ActTUpAIND_enum_maxval
      link override Signal_Limit/_minval: Value=KOUTP_ActTUpAIND_enum_minval
      link override Signal_Override/_ovrdflg: Value=KOUTP_ActTUpAIND_enum_ovrdflg
      link override Signal_Override/_ovrdval: Value=KOUTP_ActTUpAIND_enum_ovrdval
  VTQD_CreepIND_enum_Inproc : FVT_lib/outp/OverrideAndLimit  SystemSampleTime=-1  VariantActivationTime=update diagram  Latency=0  AutoFrameSizeCalculation=off
      link override Signal_Limit/_maxval: Value=KOUTP_CreepIND_enum_maxval
      link override Signal_Limit/_minval: Value=KOUTP_CreepIND_enum_minval
      link override Signal_Override/_ovrdflg: Value=KOUTP_CreepIND_enum_ovrdflg
      link override Signal_Override/_ovrdval: Value=KOUTP_CreepIND_enum_ovrdval
  VTQD_CreepSpdReq_rpm_Inproc : FVT_lib/outp/OverrideAndLimit  SystemSampleTime=-1  VariantActivationTime=update diagram  Latency=0  AutoFrameSizeCalculation=off
      link override Signal_Limit/_maxval: Value=KOUTP_CreepSpdReq_rpm_maxval
      link override Signal_Limit/_minval: Value=KOUTP_CreepSpdReq_rpm_minval
      link override Signal_Override/_ovrdflg: Value=KOUTP_CreepSpdReq_rpm_ovrdflg
      link override Signal_Override/_ovrdval: Value=KOUTP_CreepSpdReq_rpm_ovrdval
  VTQD_EC1EMDefTrqLmt_rpm_Inproc : FVT_lib/outp/OverrideAndLimit  SystemSampleTime=-1  VariantActivationTime=update diagram  Latency=0  AutoFrameSizeCalculation=off
      link override Signal_Limit/_maxval: Value=KOUTP_EC1EMDefTrqLmt_rpm_maxval
      link override Signal_Limit/_minval: Value=KOUTP_EC1EMDefTrqLmt_rpm_minval
      link override Signal_Override/_ovrdflg: Value=KOUTP_EC1EMDefTrqLmt_rpm_ovrdflg
      link override Signal_Override/_ovrdval: Value=KOUTP_EC1EMDefTrqLmt_rpm_ovrdval
  VTQD_EC1EMExtRSCtrlUpLmt_rpm_Inproc : FVT_lib/outp/OverrideAndLimit  SystemSampleTime=-1  VariantActivationTime=update diagram  Latency=0  AutoFrameSizeCalculation=off
      link override Signal_Limit/_maxval: Value=KOUTP_EC1EMExtRSCtrlUpLmt_rpm_maxval
      link override Signal_Limit/_minval: Value=KOUTP_EC1EMExtRSCtrlUpLmt_rpm_minval
      link override Signal_Override/_ovrdflg: Value=KOUTP_EC1EMExtRSCtrlUpLmt_rpm_ovrdflg
      link override Signal_Override/_ovrdval: Value=KOUTP_EC1EMExtRSCtrlUpLmt_rpm_ovrdval
  VTQD_EC1EMGainEndSpdGvn_gain_Inproc : FVT_lib/outp/OverrideAndLimit  SystemSampleTime=-1  VariantActivationTime=update diagram  Latency=0  AutoFrameSizeCalculation=off
      link override Signal_Limit/_maxval: Value=KOUTP_EC1EMGainEndSpdGvn_gain_maxval
      link override Signal_Limit/_minval: Value=KOUTP_EC1EMGainEndSpdGvn_gain_minval
      link override Signal_Override/_ovrdflg: Value=KOUTP_EC1EMGainEndSpdGvn_gain_ovrdflg
      link override Signal_Override/_ovrdval: Value=KOUTP_EC1EMGainEndSpdGvn_gain_ovrdval
  VTQD_EC1EMMaxMEngOvrSP7_rpm_Inproc : FVT_lib/outp/OverrideAndLimit  SystemSampleTime=-1  VariantActivationTime=update diagram  Latency=0  AutoFrameSizeCalculation=off
      link override Signal_Limit/_maxval: Value=KOUTP_EC1EMMaxMEngOvrSP7_rpm_maxval
      link override Signal_Limit/_minval: Value=KOUTP_EC1EMMaxMEngOvrSP7_rpm_minval
      link override Signal_Override/_ovrdflg: Value=KOUTP_EC1EMMaxMEngOvrSP7_rpm_ovrdflg
      link override Signal_Override/_ovrdval: Value=KOUTP_EC1EMMaxMEngOvrSP7_rpm_ovrdval
  VTQD_EC1EMMaxMOvrTmt_s_Inproc : FVT_lib/outp/OverrideAndLimit  SystemSampleTime=-1  VariantActivationTime=update diagram  Latency=0  AutoFrameSizeCalculation=off
      link override Signal_Limit/_maxval: Value=KOUTP_EC1EMMaxMOvrTmt_s_maxval
      link override Signal_Limit/_minval: Value=KOUTP_EC1EMMaxMOvrTmt_s_minval
      link override Signal_Override/_ovrdflg: Value=KOUTP_EC1EMMaxMOvrTmt_s_ovrdflg
      link override Signal_Override/_ovrdval: Value=KOUTP_EC1EMMaxMOvrTmt_s_ovrdval
  VTQD_EC1EMMomOfInertia_kgpm2_Inproc : FVT_lib/outp/OverrideAndLimit  SystemSampleTime=-1  VariantActivationTime=update diagram  Latency=0  AutoFrameSizeCalculation=off
      link override Signal_Limit/_maxval: Value=KOUTP_EC1EMMomOfInertia_kgpm2_maxval
      link override Signal_Limit/_minval: Value=KOUTP_EC1EMMomOfInertia_kgpm2_minval
      link override Signal_Override/_ovrdflg: Value=KOUTP_EC1EMMomOfInertia_kgpm2_ovrdflg
      link override Signal_Override/_ovrdval: Value=KOUTP_EC1EMMomOfInertia_kgpm2_ovrdval
  VTQD_EC1EMRefTorq_Nm_Inproc : FVT_lib/outp/OverrideAndLimit  SystemSampleTime=-1  VariantActivationTime=update diagram  Latency=0  AutoFrameSizeCalculation=off
      link override Signal_Limit/_maxval: Value=KOUTP_EC1EMRefTorq_Nm_maxval
      link override Signal_Limit/_minval: Value=KOUTP_EC1EMRefTorq_Nm_minval
      link override Signal_Override/_ovrdflg: Value=KOUTP_EC1EMRefTorq_Nm_ovrdflg
      link override Signal_Override/_ovrdval: Value=KOUTP_EC1EMRefTorq_Nm_ovrdval
  VTQD_EC1EMReqSpdCtrlLoLmt_rpm_Inproc : FVT_lib/outp/OverrideAndLimit  SystemSampleTime=-1  VariantActivationTime=update diagram  Latency=0  AutoFrameSizeCalculation=off
      link override Signal_Limit/_maxval: Value=KOUTP_EC1EMReqSpdCtrlLoLmt_rpm_maxval
      link override Signal_Limit/_minval: Value=KOUTP_EC1EMReqSpdCtrlLoLmt_rpm_minval
      link override Signal_Override/_ovrdflg: Value=KOUTP_EC1EMReqSpdCtrlLoLmt_rpm_ovrdflg
      link override Signal_Override/_ovrdval: Value=KOUTP_EC1EMReqSpdCtrlLoLmt_rpm_ovrdval
  VTQD_EC1EMReqSpdCtrlUpLmt_rpm_Inproc : FVT_lib/outp/OverrideAndLimit  SystemSampleTime=-1  VariantActivationTime=update diagram  Latency=0  AutoFrameSizeCalculation=off
      link override Signal_Limit/_maxval: Value=KOUTP_EC1EMReqSpdCtrlUpLmt_rpm_maxval
      link override Signal_Limit/_minval: Value=KOUTP_EC1EMReqSpdCtrlUpLmt_rpm_minval
      link override Signal_Override/_ovrdflg: Value=KOUTP_EC1EMReqSpdCtrlUpLmt_rpm_ovrdflg
      link override Signal_Override/_ovrdval: Value=KOUTP_EC1EMReqSpdCtrlUpLmt_rpm_ovrdval
  VTQD_EC1EMReqTrqCtrlLoLmt_pct_Inproc : FVT_lib/outp/OverrideAndLimit  SystemSampleTime=-1  VariantActivationTime=update diagram  Latency=0  AutoFrameSizeCalculation=off
      link override Signal_Limit/_maxval: Value=KOUTP_EC1EMReqTrqCtrlLoLmt_pct_maxval
      link override Signal_Limit/_minval: Value=KOUTP_EC1EMReqTrqCtrlLoLmt_pct_minval
      link override Signal_Override/_ovrdflg: Value=KOUTP_EC1EMReqTrqCtrlLoLmt_pct_ovrdflg
      link override Signal_Override/_ovrdval: Value=KOUTP_EC1EMReqTrqCtrlLoLmt_pct_ovrdval
  VTQD_EC1EMReqTrqCtrlUpLmt_pct_Inproc : FVT_lib/outp/OverrideAndLimit  SystemSampleTime=-1  VariantActivationTime=update diagram  Latency=0  AutoFrameSizeCalculation=off
      link override Signal_Limit/_maxval: Value=KOUTP_EC1EMReqTrqCtrlUpLmt_pct_maxval
      link override Signal_Limit/_minval: Value=KOUTP_EC1EMReqTrqCtrlUpLmt_pct_minval
      link override Signal_Override/_ovrdflg: Value=KOUTP_EC1EMReqTrqCtrlUpLmt_pct_ovrdflg
      link override Signal_Override/_ovrdval: Value=KOUTP_EC1EMReqTrqCtrlUpLmt_pct_ovrdval
  VTQD_EC1EMSpdHdleP6_rpm_Inproc : FVT_lib/outp/OverrideAndLimit  SystemSampleTime=-1  VariantActivationTime=update diagram  Latency=0  AutoFrameSizeCalculation=off
      link override Signal_Limit/_maxval: Value=KOUTP_EC1EMSpdHdleP6_rpm_maxval
      link override Signal_Limit/_minval: Value=KOUTP_EC1EMSpdHdleP6_rpm_minval
      link override Signal_Override/_ovrdflg: Value=KOUTP_EC1EMSpdHdleP6_rpm_ovrdflg
      link override Signal_Override/_ovrdval: Value=KOUTP_EC1EMSpdHdleP6_rpm_ovrdval
  VTQD_EC1EMSpdIdleP1_rpm_Inproc : FVT_lib/outp/OverrideAndLimit  SystemSampleTime=-1  VariantActivationTime=update diagram  Latency=0  AutoFrameSizeCalculation=off
      link override Signal_Limit/_maxval: Value=KOUTP_EC1EMSpdIdleP1_rpm_maxval
      link override Signal_Limit/_minval: Value=KOUTP_EC1EMSpdIdleP1_rpm_minval
      link override Signal_Override/_ovrdflg: Value=KOUTP_EC1EMSpdIdleP1_rpm_ovrdflg
      link override Signal_Override/_ovrdval: Value=KOUTP_EC1EMSpdIdleP1_rpm_ovrdval
  VTQD_EC1EMSpdIdleP2_rpm_Inproc : FVT_lib/outp/OverrideAndLimit  SystemSampleTime=-1  VariantActivationTime=update diagram  Latency=0  AutoFrameSizeCalculation=off
      link override Signal_Limit/_maxval: Value=KOUTP_EC1EMSpdIdleP2_rpm_maxval
      link override Signal_Limit/_minval: Value=KOUTP_EC1EMSpdIdleP2_rpm_minval
      link override Signal_Override/_ovrdflg: Value=KOUTP_EC1EMSpdIdleP2_rpm_ovrdflg
      link override Signal_Override/_ovrdval: Value=KOUTP_EC1EMSpdIdleP2_rpm_ovrdval
  VTQD_EC1EMSpdIdleP3_rpm_Inproc : FVT_lib/outp/OverrideAndLimit  SystemSampleTime=-1  VariantActivationTime=update diagram  Latency=0  AutoFrameSizeCalculation=off
      link override Signal_Limit/_maxval: Value=KOUTP_EC1EMSpdIdleP3_rpm_maxval
      link override Signal_Limit/_minval: Value=KOUTP_EC1EMSpdIdleP3_rpm_minval
      link override Signal_Override/_ovrdflg: Value=KOUTP_EC1EMSpdIdleP3_rpm_ovrdflg
      link override Signal_Override/_ovrdval: Value=KOUTP_EC1EMSpdIdleP3_rpm_ovrdval
  VTQD_EC1EMSpdIdleP4_rpm_Inproc : FVT_lib/outp/OverrideAndLimit  SystemSampleTime=-1  VariantActivationTime=update diagram  Latency=0  AutoFrameSizeCalculation=off
      link override Signal_Limit/_maxval: Value=KOUTP_EC1EMSpdIdleP4_rpm_maxval
      link override Signal_Limit/_minval: Value=KOUTP_EC1EMSpdIdleP4_rpm_minval
      link override Signal_Override/_ovrdflg: Value=KOUTP_EC1EMSpdIdleP4_rpm_ovrdflg
      link override Signal_Override/_ovrdval: Value=KOUTP_EC1EMSpdIdleP4_rpm_ovrdval
  VTQD_EC1EMSpdIdleP5_rpm_Inproc : FVT_lib/outp/OverrideAndLimit  SystemSampleTime=-1  VariantActivationTime=update diagram  Latency=0  AutoFrameSizeCalculation=off
      link override Signal_Limit/_maxval: Value=KOUTP_EC1EMSpdIdleP5_rpm_maxval
      link override Signal_Limit/_minval: Value=KOUTP_EC1EMSpdIdleP5_rpm_minval
      link override Signal_Override/_ovrdflg: Value=KOUTP_EC1EMSpdIdleP5_rpm_ovrdflg
      link override Signal_Override/_ovrdval: Value=KOUTP_EC1EMSpdIdleP5_rpm_ovrdval
  VTQD_EC1EMSupTSC1CtrlPG1_cnt_Inproc : FVT_lib/outp/OverrideAndLimit  SystemSampleTime=-1  VariantActivationTime=update diagram  Latency=0  AutoFrameSizeCalculation=off
      link override Signal_Limit/_maxval: Value=KOUTP_EC1EMSupTSC1CtrlPG1_cnt_maxval
      link override Signal_Limit/_minval: Value=KOUTP_EC1EMSupTSC1CtrlPG1_cnt_minval
      link override Signal_Override/_ovrdflg: Value=KOUTP_EC1EMSupTSC1CtrlPG1_cnt_ovrdflg
      link override Signal_Override/_ovrdval: Value=KOUTP_EC1EMSupTSC1CtrlPG1_cnt_ovrdval
  VTQD_EC1EMSupTSC1CtrlPG2_cnt_Inproc : FVT_lib/outp/OverrideAndLimit  SystemSampleTime=-1  VariantActivationTime=update diagram  Latency=0  AutoFrameSizeCalculation=off
      link override Signal_Limit/_maxval: Value=KOUTP_EC1EMSupTSC1CtrlPG2_cnt_maxval
      link override Signal_Limit/_minval: Value=KOUTP_EC1EMSupTSC1CtrlPG2_cnt_minval
      link override Signal_Override/_ovrdflg: Value=KOUTP_EC1EMSupTSC1CtrlPG2_cnt_ovrdflg
      link override Signal_Override/_ovrdval: Value=KOUTP_EC1EMSupTSC1CtrlPG2_cnt_ovrdval
  VTQD_EC1EMSupTSC1CtrlPG3_cnt_Inproc : FVT_lib/outp/OverrideAndLimit  SystemSampleTime=-1  VariantActivationTime=update diagram  Latency=0  AutoFrameSizeCalculation=off
      link override Signal_Limit/_maxval: Value=KOUTP_EC1EMSupTSC1CtrlPG3_cnt_maxval
      link override Signal_Limit/_minval: Value=KOUTP_EC1EMSupTSC1CtrlPG3_cnt_minval
      link override Signal_Override/_ovrdflg: Value=KOUTP_EC1EMSupTSC1CtrlPG3_cnt_ovrdflg
      link override Signal_Override/_ovrdval: Value=KOUTP_EC1EMSupTSC1CtrlPG3_cnt_ovrdval
  VTQD_EC1EMSupTSC1CtrlPG4_cnt_Inproc : FVT_lib/outp/OverrideAndLimit  SystemSampleTime=-1  VariantActivationTime=update diagram  Latency=0  AutoFrameSizeCalculation=off
      link override Signal_Limit/_maxval: Value=KOUTP_EC1EMSupTSC1CtrlPG4_cnt_maxval
      link override Signal_Limit/_minval: Value=KOUTP_EC1EMSupTSC1CtrlPG4_cnt_minval
      link override Signal_Override/_ovrdflg: Value=KOUTP_EC1EMSupTSC1CtrlPG4_cnt_ovrdflg
      link override Signal_Override/_ovrdval: Value=KOUTP_EC1EMSupTSC1CtrlPG4_cnt_ovrdval
  VTQD_EC1EMSupVarRTSC1MSG_cnt_Inproc : FVT_lib/outp/OverrideAndLimit  SystemSampleTime=-1  VariantActivationTime=update diagram  Latency=0  AutoFrameSizeCalculation=off
      link override Signal_Limit/_maxval: Value=KOUTP_EC1EMSupVarRTSC1MSG_cnt_maxval
      link override Signal_Limit/_minval: Value=KOUTP_EC1EMSupVarRTSC1MSG_cnt_minval
